simulink library "ammclib_bam_S32K3xx"  (R2016a)
(part 15 of 50)

      |     warning(['Parameter u16NShift_D of ' gcb ' exceeds the fixed-point range.']);
      |   end
      |   u16NShift_Q=ceil(log2(abs(cc1fq)));
      |   tmpsh=ceil(log2(abs(cc2fq)));
      |   if u16NShift_Q<tmpsh
      |     u16NShift_Q=tmpsh;
      |   end
      |   if u16NShift_Q<0
      |     u16NShift_Q=0;
      |   end
      |   if u16NShift_Q>31
      |     u16NShift_Q=31;
      |     warning(['Parameter u16NShift_Q of ' gcb ' exceeds the fixed-point range.']);
      |   end
      |   f32CC1sc_D=round(cc1fd*2^(-u16NShift_D)*2^31);
      |   if f32CC1sc_D>2^31-1
      |     f32CC1sc_D=2^31-1;
      |     warning(['Parameter f32CC1sc_D of ' gcb ' exceeds the fixed-point range.']);
      |   end
      |   if f32CC1sc_D<-2^31
      |     f32CC1sc_D=-2^31;
      |     warning(['Parameter f32CC1sc_D of ' gcb ' exceeds the fixed-point range.']);
      |   end
      |   f32CC2sc_D=round(cc2fd*2^(-u16NShift_D)*2^31);
      |   if f32CC2sc_D>2^31-1
      |     f32CC2sc_D=2^31-1;
      |     warning(['Parameter f32CC2sc_D of ' gcb ' exceeds the fixed-point range.']);
      |   end
      |   if f32CC2sc_D<-2^31
      |     f32CC2sc_D=-2^31;
      |     warning(['Parameter f32CC2sc_D of ' gcb ' exceeds the fixed-point range.']);
      |   end
      |   f32CC1sc_Q=round(cc1fq*2^(-u16NShift_Q)*2^31);
      |   if f32CC1sc_Q>2^31-1
      |     f32CC1sc_Q=2^31-1;
      |     warning(['Parameter f32CC1sc_Q of ' gcb ' exceeds the fixed-point range.']);
      |   end
      |   if f32CC1sc_Q<-2^31
      |     f32CC1sc_Q=-2^31;
      |     warning(['Parameter f32CC1sc_Q of ' gcb ' exceeds the fixed-point range.']);
      |   end
      |   f32CC2sc_Q=round(cc2fq*2^(-u16NShift_Q)*2^31);
      |   if f32CC2sc_Q>2^31-1
      |     f32CC2sc_Q=2^31-1;
      |     warning(['Parameter f32CC2sc_Q of ' gcb ' exceeds the fixed-point range.']);
      |   end
      |   if f32CC2sc_Q<-2^31
      |     f32CC2sc_Q=-2^31;
      |     warning(['Parameter f32CC2sc_Q of ' gcb ' exceeds the fixed-point range.']);
      |   end
      |   if isnan(f32CC1sc_D)
      |     if ~strcmp(f32CC1sc_D_bkup,'0')
      |       set_param(gcb,'f32CC1sc_D','0');
      |     end
      |   else
      |     tmps=num2str(f32CC1sc_D);
      |     if ~strcmp(f32CC1sc_D_bkup,tmps)
      |       set_param(gcb,'f32CC1sc_D',tmps);
      |     end
      |   end
      |   if isnan(f32CC2sc_D)
      |     if ~strcmp(f32CC2sc_D_bkup,'0')
      |       set_param(gcb,'f32CC2sc_D','0');
      |     end
      |   else
      |     tmps=num2str(f32CC2sc_D);
      |     if ~strcmp(f32CC2sc_D_bkup,tmps)
      |       set_param(gcb,'f32CC2sc_D',tmps);
      |     end
      |   end
      |   if isnan(u16NShift_D)
      |     if ~strcmp(u16NShift_D_bkup,'0')
      |       set_param(gcb,'u16NShift_D','0');
      |     end
      |   else
      |     tmps=num2str(u16NShift_D);
      |     if ~strcmp(u16NShift_D_bkup,tmps)
      |       set_param(gcb,'u16NShift_D',tmps);
      |     end
      |   end
      |   if isnan(f32CC1sc_Q)
      |     if ~strcmp(f32CC1sc_Q_bkup,'0')
      |       set_param(gcb,'f32CC1sc_Q','0');
      |     end
      |   else
      |     tmps=num2str(f32CC1sc_Q);
      |     if ~strcmp(f32CC1sc_Q_bkup,tmps)
      |       set_param(gcb,'f32CC1sc_Q',tmps);
      |     end
      |   end
      |   if isnan(f32CC2sc_Q)
      |     if ~strcmp(f32CC2sc_Q_bkup,'0')
      |       set_param(gcb,'f32CC2sc_Q','0');
      |     end
      |   else
      |     tmps=num2str(f32CC2sc_Q);
      |     if ~strcmp(f32CC2sc_Q_bkup,tmps)
      |       set_param(gcb,'f32CC2sc_Q',tmps);
      |     end
      |   end
      |   if isnan(u16NShift_Q)
      |     if ~strcmp(u16NShift_Q_bkup,'0')
      |       set_param(gcb,'u16NShift_Q','0');
      |     end
      |   else
      |     tmps=num2str(u16NShift_Q);
      |     if ~strcmp(u16NShift_Q_bkup,tmps)
      |       set_param(gcb,'u16NShift_Q',tmps);
      |     end
      |   end
      | end
      mask Callback iscale:
      | autoCalcEn=get_param(gcb,'autoCalcEn');
      | if strcmp(autoCalcEn,'on')
      |   SampleTime=Simulink.data.evalinGlobal(bdroot,get_param(gcb,'SampleTime'));
      |   if (SampleTime==-1)
      |     SampleTime=str2double(get_param(gcb,'SampleTime_1'));
      |   end
      |   f32CC1sc_D_bkup=get_param(gcb,'f32CC1sc_D');
      |   f32CC2sc_D_bkup=get_param(gcb,'f32CC2sc_D');
      |   u16NShift_D_bkup=get_param(gcb,'u16NShift_D');
      |   f32CC1sc_Q_bkup=get_param(gcb,'f32CC1sc_Q');
      |   f32CC2sc_Q_bkup=get_param(gcb,'f32CC2sc_Q');
      |   u16NShift_Q_bkup=get_param(gcb,'u16NShift_Q');
      |   intmethod=get_param(gcb,'intmethod');
      |   if0=Simulink.data.evalinGlobal(bdroot,get_param(gcb,'if0'));
      |   iksi=Simulink.data.evalinGlobal(bdroot,get_param(gcb,'iksi'));
      |   Ld=Simulink.data.evalinGlobal(bdroot,get_param(gcb,'Ld'));
      |   Lq=Simulink.data.evalinGlobal(bdroot,get_param(gcb,'Lq'));
      |   Rs=Simulink.data.evalinGlobal(bdroot,get_param(gcb,'Rs'));
      |   uscale=Simulink.data.evalinGlobal(bdroot,get_param(gcb,'uscale'));
      |   iscale=Simulink.data.evalinGlobal(bdroot,get_param(gcb,'iscale'));
      |   if (if0<=0)
      |     warning('Natural frequency f0 must be positive.');
      |   end
      |   if (iksi<=0)
      |     warning('Current loop attenuation must be positive.');
      |   end
      |   if (iksi>1)
      |     warning('Current loop attenuation must not exceed 1.');
      |   end
      |   if (Ld<=0)
      |     warning('Inductance Ld must be positive.');
      |   end
      |   if (Lq<=0)
      |     warning('Inductance Lq must be positive.');
      |   end
      |   if (Rs<0)
      |     warning('Resistance Rs must be non-negative.');
      |   end
      |   if (uscale<=0)
      |     warning('U_max must be positive.');
      |   end
      |   if (iscale<=0)
      |     warning('I_max must be positive.');
      |   end
      |   w0=6.283185307179586*if0;
      |   pgainD=2.0*iksi*w0*Ld-Rs;
      |   igainD=w0*w0*Ld;
      |   pgainQ=2.0*iksi*w0*Lq-Rs;
      |   igainQ=w0*w0*Lq;
      |   if strcmp(intmethod,'Forward Rectangular')
      |     cc1d=pgainD;
      |     cc2d=-pgainD+igainD*SampleTime;
      |     cc1q=pgainQ;
      |     cc2q=-pgainQ+igainQ*SampleTime;
      |   else
      |     if strcmp(intmethod,'Backward Rectangular')
      |       cc1d=pgainD+igainD*SampleTime;
      |       cc2d=-pgainD;
      |       cc1q=pgainQ+igainQ*SampleTime;
      |       cc2q=-pgainQ;
      |     else
      |       cc1d=pgainD+igainD*SampleTime*0.5;
      |       cc2d=-pgainD+igainD*SampleTime*0.5;
      |       cc1q=pgainQ+igainQ*SampleTime*0.5;
      |       cc2q=-pgainQ+igainQ*SampleTime*0.5;
      |     end
      |   end
      |   cc1fd=cc1d*iscale/uscale;
      |   cc2fd=cc2d*iscale/uscale;
      |   cc1fq=cc1q*iscale/uscale;
      |   cc2fq=cc2q*iscale/uscale;
      |   u16NShift_D=ceil(log2(abs(cc1fd)));
      |   tmpsh=ceil(log2(abs(cc2fd)));
      |   if u16NShift_D<tmpsh
      |     u16NShift_D=tmpsh;
      |   end
      |   if u16NShift_D<0
      |     u16NShift_D=0;
      |   end
      |   if u16NShift_D>31
      |     u16NShift_D=31;
      |     warning(['Parameter u16NShift_D of ' gcb ' exceeds the fixed-point range.']);
      |   end
      |   u16NShift_Q=ceil(log2(abs(cc1fq)));
      |   tmpsh=ceil(log2(abs(cc2fq)));
      |   if u16NShift_Q<tmpsh
      |     u16NShift_Q=tmpsh;
      |   end
      |   if u16NShift_Q<0
      |     u16NShift_Q=0;
      |   end
      |   if u16NShift_Q>31
      |     u16NShift_Q=31;
      |     warning(['Parameter u16NShift_Q of ' gcb ' exceeds the fixed-point range.']);
      |   end
      |   f32CC1sc_D=round(cc1fd*2^(-u16NShift_D)*2^31);
      |   if f32CC1sc_D>2^31-1
      |     f32CC1sc_D=2^31-1;
      |     warning(['Parameter f32CC1sc_D of ' gcb ' exceeds the fixed-point range.']);
      |   end
      |   if f32CC1sc_D<-2^31
      |     f32CC1sc_D=-2^31;
      |     warning(['Parameter f32CC1sc_D of ' gcb ' exceeds the fixed-point range.']);
      |   end
      |   f32CC2sc_D=round(cc2fd*2^(-u16NShift_D)*2^31);
      |   if f32CC2sc_D>2^31-1
      |     f32CC2sc_D=2^31-1;
      |     warning(['Parameter f32CC2sc_D of ' gcb ' exceeds the fixed-point range.']);
      |   end
      |   if f32CC2sc_D<-2^31
      |     f32CC2sc_D=-2^31;
      |     warning(['Parameter f32CC2sc_D of ' gcb ' exceeds the fixed-point range.']);
      |   end
      |   f32CC1sc_Q=round(cc1fq*2^(-u16NShift_Q)*2^31);
      |   if f32CC1sc_Q>2^31-1
      |     f32CC1sc_Q=2^31-1;
      |     warning(['Parameter f32CC1sc_Q of ' gcb ' exceeds the fixed-point range.']);
      |   end
      |   if f32CC1sc_Q<-2^31
      |     f32CC1sc_Q=-2^31;
      |     warning(['Parameter f32CC1sc_Q of ' gcb ' exceeds the fixed-point range.']);
      |   end
      |   f32CC2sc_Q=round(cc2fq*2^(-u16NShift_Q)*2^31);
      |   if f32CC2sc_Q>2^31-1
      |     f32CC2sc_Q=2^31-1;
      |     warning(['Parameter f32CC2sc_Q of ' gcb ' exceeds the fixed-point range.']);
      |   end
      |   if f32CC2sc_Q<-2^31
      |     f32CC2sc_Q=-2^31;
      |     warning(['Parameter f32CC2sc_Q of ' gcb ' exceeds the fixed-point range.']);
      |   end
      |   if isnan(f32CC1sc_D)
      |     if ~strcmp(f32CC1sc_D_bkup,'0')
      |       set_param(gcb,'f32CC1sc_D','0');
      |     end
      |   else
      |     tmps=num2str(f32CC1sc_D);
      |     if ~strcmp(f32CC1sc_D_bkup,tmps)
      |       set_param(gcb,'f32CC1sc_D',tmps);
      |     end
      |   end
      |   if isnan(f32CC2sc_D)
      |     if ~strcmp(f32CC2sc_D_bkup,'0')
      |       set_param(gcb,'f32CC2sc_D','0');
      |     end
      |   else
      |     tmps=num2str(f32CC2sc_D);
      |     if ~strcmp(f32CC2sc_D_bkup,tmps)
      |       set_param(gcb,'f32CC2sc_D',tmps);
      |     end
      |   end
      |   if isnan(u16NShift_D)
      |     if ~strcmp(u16NShift_D_bkup,'0')
      |       set_param(gcb,'u16NShift_D','0');
      |     end
      |   else
      |     tmps=num2str(u16NShift_D);
      |     if ~strcmp(u16NShift_D_bkup,tmps)
      |       set_param(gcb,'u16NShift_D',tmps);
      |     end
      |   end
      |   if isnan(f32CC1sc_Q)
      |     if ~strcmp(f32CC1sc_Q_bkup,'0')
      |       set_param(gcb,'f32CC1sc_Q','0');
      |     end
      |   else
      |     tmps=num2str(f32CC1sc_Q);
      |     if ~strcmp(f32CC1sc_Q_bkup,tmps)
      |       set_param(gcb,'f32CC1sc_Q',tmps);
      |     end
      |   end
      |   if isnan(f32CC2sc_Q)
      |     if ~strcmp(f32CC2sc_Q_bkup,'0')
      |       set_param(gcb,'f32CC2sc_Q','0');
      |     end
      |   else
      |     tmps=num2str(f32CC2sc_Q);
      |     if ~strcmp(f32CC2sc_Q_bkup,tmps)
      |       set_param(gcb,'f32CC2sc_Q',tmps);
      |     end
      |   end
      |   if isnan(u16NShift_Q)
      |     if ~strcmp(u16NShift_Q_bkup,'0')
      |       set_param(gcb,'u16NShift_Q','0');
      |     end
      |   else
      |     tmps=num2str(u16NShift_Q);
      |     if ~strcmp(u16NShift_Q_bkup,tmps)
      |       set_param(gcb,'u16NShift_Q',tmps);
      |     end
      |   end
      | end
      mask Callback autoCalcEn:
      | maskStr=get_param(gcb,'showStates');
      | if strcmp(maskStr,'Hide (faster execution)')
      |   p=Simulink.Mask.get(gcb);
      |   autoCalcEn=get_param(gcb,'autoCalcEn');
      |   hintText=p.getDialogControl('timeHint');
      |   if strcmp(autoCalcEn,'on')
      |     param=p.getParameter('iscale');
      |     if strcmp(param.Enabled,'off')
      |       SampleTime=Simulink.data.evalinGlobal(bdroot,get_param(gcb,'SampleTime'));
      |       if SampleTime==-1
      |         SampleTime=str2double(get_param(gcb,'SampleTime_1'));
      |         if isnan(SampleTime)
      |           hintText.Prompt=['Note: Implementation parameters cannot be calculated yet because the block''s inherited sample time is unknown. Simulink will update the sample time when you run the simulation.'];
      |         else
      |           hintText.Prompt=['Caution: Implementation parameters depend on inherited sample time. Make sure that the sample time of the block''s inputs corresponds to the sampling period in the target application.'];
      |         end
      |       else
      |         hintText.Prompt='Caution: Implementation parameters depend on the sample time. Make sure that the simulation time step corresponds to the sampling period in the target application.';
      |       end
      |       p=Simulink.Mask.get(gcb);
      |       param=p.getParameter('intmethod');
      |       param.set('Enabled','on');
      |       param=p.getParameter('if0');
      |       param.set('Enabled','on');
      |       param=p.getParameter('iksi');
      |       param.set('Enabled','on');
      |       param=p.getParameter('Ld');
      |       param.set('Enabled','on');
      |       param=p.getParameter('Lq');
      |       param.set('Enabled','on');
      |       param=p.getParameter('Rs');
      |       param.set('Enabled','on');
      |       param=p.getParameter('uscale');
      |       param.set('Enabled','on');
      |       param=p.getParameter('iscale');
      |       param.set('Enabled','on');
      |     else
      |       SampleTime=Simulink.data.evalinGlobal(bdroot,get_param(gcb,'SampleTime'));
      |       if SampleTime==-1
      |         SampleTime=str2double(get_param(gcb,'SampleTime_1'));
      |       end
      |     end
      |     f32CC1sc_D_bkup=get_param(gcb,'f32CC1sc_D');
      |     f32CC2sc_D_bkup=get_param(gcb,'f32CC2sc_D');
      |     u16NShift_D_bkup=get_param(gcb,'u16NShift_D');
      |     f32CC1sc_Q_bkup=get_param(gcb,'f32CC1sc_Q');
      |     f32CC2sc_Q_bkup=get_param(gcb,'f32CC2sc_Q');
      |     u16NShift_Q_bkup=get_param(gcb,'u16NShift_Q');
      |     intmethod=get_param(gcb,'intmethod');
      |     if0=Simulink.data.evalinGlobal(bdroot,get_param(gcb,'if0'));
      |     iksi=Simulink.data.evalinGlobal(bdroot,get_param(gcb,'iksi'));
      |     Ld=Simulink.data.evalinGlobal(bdroot,get_param(gcb,'Ld'));
      |     Lq=Simulink.data.evalinGlobal(bdroot,get_param(gcb,'Lq'));
      |     Rs=Simulink.data.evalinGlobal(bdroot,get_param(gcb,'Rs'));
      |     uscale=Simulink.data.evalinGlobal(bdroot,get_param(gcb,'uscale'));
      |     iscale=Simulink.data.evalinGlobal(bdroot,get_param(gcb,'iscale'));
      |     if (if0<=0)
      |       warning('Natural frequency f0 must be positive.');
      |     end
      |     if (iksi<=0)
      |       warning('Current loop attenuation must be positive.');
      |     end
      |     if (iksi>1)
      |       warning('Current loop attenuation must not exceed 1.');
      |     end
      |     if (Ld<=0)
      |       warning('Inductance Ld must be positive.');
      |     end
      |     if (Lq<=0)
      |       warning('Inductance Lq must be positive.');
      |     end
      |     if (Rs<0)
      |       warning('Resistance Rs must be non-negative.');
      |     end
      |     if (uscale<=0)
      |       warning('U_max must be positive.');
      |     end
      |     if (iscale<=0)
      |       warning('I_max must be positive.');
      |     end
      |     w0=6.283185307179586*if0;
      |     pgainD=2.0*iksi*w0*Ld-Rs;
      |     igainD=w0*w0*Ld;
      |     pgainQ=2.0*iksi*w0*Lq-Rs;
      |     igainQ=w0*w0*Lq;
      |     if strcmp(intmethod,'Forward Rectangular')
      |       cc1d=pgainD;
      |       cc2d=-pgainD+igainD*SampleTime;
      |       cc1q=pgainQ;
      |       cc2q=-pgainQ+igainQ*SampleTime;
      |     else
      |       if strcmp(intmethod,'Backward Rectangular')
      |         cc1d=pgainD+igainD*SampleTime;
      |         cc2d=-pgainD;
      |         cc1q=pgainQ+igainQ*SampleTime;
      |         cc2q=-pgainQ;
      |       else
      |         cc1d=pgainD+igainD*SampleTime*0.5;
      |         cc2d=-pgainD+igainD*SampleTime*0.5;
      |         cc1q=pgainQ+igainQ*SampleTime*0.5;
      |         cc2q=-pgainQ+igainQ*SampleTime*0.5;
      |       end
      |     end
      |     cc1fd=cc1d*iscale/uscale;
      |     cc2fd=cc2d*iscale/uscale;
      |     cc1fq=cc1q*iscale/uscale;
      |     cc2fq=cc2q*iscale/uscale;
      |     u16NShift_D=ceil(log2(abs(cc1fd)));
      |     tmpsh=ceil(log2(abs(cc2fd)));
      |     if u16NShift_D<tmpsh
      |       u16NShift_D=tmpsh;
      |     end
      |     if u16NShift_D<0
      |       u16NShift_D=0;
      |     end
      |     if u16NShift_D>31
      |       u16NShift_D=31;
      |       warning(['Parameter u16NShift_D of ' gcb ' exceeds the fixed-point range.']);
      |     end
      |     u16NShift_Q=ceil(log2(abs(cc1fq)));
      |     tmpsh=ceil(log2(abs(cc2fq)));
      |     if u16NShift_Q<tmpsh
      |       u16NShift_Q=tmpsh;
      |     end
      |     if u16NShift_Q<0
      |       u16NShift_Q=0;
      |     end
      |     if u16NShift_Q>31
      |       u16NShift_Q=31;
      |       warning(['Parameter u16NShift_Q of ' gcb ' exceeds the fixed-point range.']);
      |     end
      |     f32CC1sc_D=round(cc1fd*2^(-u16NShift_D)*2^31);
      |     if f32CC1sc_D>2^31-1
      |       f32CC1sc_D=2^31-1;
      |       warning(['Parameter f32CC1sc_D of ' gcb ' exceeds the fixed-point range.']);
      |     end
      |     if f32CC1sc_D<-2^31
      |       f32CC1sc_D=-2^31;
      |       warning(['Parameter f32CC1sc_D of ' gcb ' exceeds the fixed-point range.']);
      |     end
      |     f32CC2sc_D=round(cc2fd*2^(-u16NShift_D)*2^31);
      |     if f32CC2sc_D>2^31-1
      |       f32CC2sc_D=2^31-1;
      |       warning(['Parameter f32CC2sc_D of ' gcb ' exceeds the fixed-point range.']);
      |     end
      |     if f32CC2sc_D<-2^31
      |       f32CC2sc_D=-2^31;
      |       warning(['Parameter f32CC2sc_D of ' gcb ' exceeds the fixed-point range.']);
      |     end
      |     f32CC1sc_Q=round(cc1fq*2^(-u16NShift_Q)*2^31);
      |     if f32CC1sc_Q>2^31-1
      |       f32CC1sc_Q=2^31-1;
      |       warning(['Parameter f32CC1sc_Q of ' gcb ' exceeds the fixed-point range.']);
      |     end
      |     if f32CC1sc_Q<-2^31
      |       f32CC1sc_Q=-2^31;
      |       warning(['Parameter f32CC1sc_Q of ' gcb ' exceeds the fixed-point range.']);
      |     end
      |     f32CC2sc_Q=round(cc2fq*2^(-u16NShift_Q)*2^31);
      |     if f32CC2sc_Q>2^31-1
      |       f32CC2sc_Q=2^31-1;
      |       warning(['Parameter f32CC2sc_Q of ' gcb ' exceeds the fixed-point range.']);
      |     end
      |     if f32CC2sc_Q<-2^31
      |       f32CC2sc_Q=-2^31;
      |       warning(['Parameter f32CC2sc_Q of ' gcb ' exceeds the fixed-point range.']);
      |     end
      |     if isnan(f32CC1sc_D)
      |       if ~strcmp(f32CC1sc_D_bkup,'0')
      |         set_param(gcb,'f32CC1sc_D','0');
      |       end
      |     else
      |       tmps=num2str(f32CC1sc_D);
      |       if ~strcmp(f32CC1sc_D_bkup,tmps)
      |         set_param(gcb,'f32CC1sc_D',tmps);
      |       end
      |     end
      |     if isnan(f32CC2sc_D)
      |       if ~strcmp(f32CC2sc_D_bkup,'0')
      |         set_param(gcb,'f32CC2sc_D','0');
      |       end
      |     else
      |       tmps=num2str(f32CC2sc_D);
      |       if ~strcmp(f32CC2sc_D_bkup,tmps)
      |         set_param(gcb,'f32CC2sc_D',tmps);
      |       end
      |     end
      |     if isnan(u16NShift_D)
      |       if ~strcmp(u16NShift_D_bkup,'0')
      |         set_param(gcb,'u16NShift_D','0');
      |       end
      |     else
      |       tmps=num2str(u16NShift_D);
      |       if ~strcmp(u16NShift_D_bkup,tmps)
      |         set_param(gcb,'u16NShift_D',tmps);
      |       end
      |     end
      |     if isnan(f32CC1sc_Q)
      |       if ~strcmp(f32CC1sc_Q_bkup,'0')
      |         set_param(gcb,'f32CC1sc_Q','0');
      |       end
      |     else
      |       tmps=num2str(f32CC1sc_Q);
      |       if ~strcmp(f32CC1sc_Q_bkup,tmps)
      |         set_param(gcb,'f32CC1sc_Q',tmps);
      |       end
      |     end
      |     if isnan(f32CC2sc_Q)
      |       if ~strcmp(f32CC2sc_Q_bkup,'0')
      |         set_param(gcb,'f32CC2sc_Q','0');
      |       end
      |     else
      |       tmps=num2str(f32CC2sc_Q);
      |       if ~strcmp(f32CC2sc_Q_bkup,tmps)
      |         set_param(gcb,'f32CC2sc_Q',tmps);
      |       end
      |     end
      |     if isnan(u16NShift_Q)
      |       if ~strcmp(u16NShift_Q_bkup,'0')
      |         set_param(gcb,'u16NShift_Q','0');
      |       end
      |     else
      |       tmps=num2str(u16NShift_Q);
      |       if ~strcmp(u16NShift_Q_bkup,tmps)
      |         set_param(gcb,'u16NShift_Q',tmps);
      |       end
      |     end
      |   else
      |     param=p.getParameter('iscale');
      |     if strcmp(param.Enabled,'on')
      |       hintText.Prompt='Caution: Implementation parameters are fixed.';
      |       p=Simulink.Mask.get(gcb);
      |       param=p.getParameter('intmethod');
      |       param.set('Enabled','off');
      |       param=p.getParameter('if0');
      |       param.set('Enabled','off');
      |       param=p.getParameter('iksi');
      |       param.set('Enabled','off');
      |       param=p.getParameter('Ld');
      |       param.set('Enabled','off');
      |       param=p.getParameter('Lq');
      |       param.set('Enabled','off');
      |       param=p.getParameter('Rs');
      |       param.set('Enabled','off');
      |       param=p.getParameter('uscale');
      |       param.set('Enabled','off');
      |       param=p.getParameter('iscale');
      |       param.set('Enabled','off');
      |     end
      |   end
      | end
      mask DialogControl CompBut Prompt: Recalculate sample times
      mask DialogControl CompBut Tooltip: Simulink updates the sample times of all blocks when the simulation is run. This button will update the sample times now.
      mask DialogControl CompBut Callback:
      | btn=questdlg('This will apply all changes in all open dialog boxes and update the schematic. Do you want to proceed?','Apply all changes','Continue','Cancel','Continue');
      | if strcmp(btn,'Continue')
      |   dlgs=DAStudio.ToolRoot.getOpenDialogs;
      |   for i=1:length(dlgs)
      |     dlgs(i).apply;
      |   end
      |   try
      |     SampleTime_1=str2double(get_param(gcb,'SampleTime_1'));
      |     ts=Simulink.Block.getSampleTimes(gcb);
      |     ts=ts(1).Value(1);
      |     if (SampleTime_1 ~= ts)
      |       SampleTime_1=ts;
      |       set_param(gcb,'SampleTime_1',num2str(ts));
      |       autoCalcEn=get_param(gcb,'autoCalcEn');
      |       if strcmp(autoCalcEn,'on')
      |         SampleTime=Simulink.data.evalinGlobal(bdroot,get_param(gcb,'SampleTime'));
      |         p=Simulink.Mask.get(gcb);
      |         hintText=p.getDialogControl('timeHint');
      |         if SampleTime==-1
      |           SampleTime=SampleTime_1;
      |           hintText.Prompt='Caution: Implementation parameters depend on inherited sample time. Make sure that the sample time of the block''s inputs corresponds to the sampling period in the target application.';
      |         else
      |           hintText.Prompt='Caution: Implementation parameters depend on the sample time. Make sure that the simulation time step corresponds to the sampling period in the target application.';
      |         end
      |         f32CC1sc_D_bkup=get_param(gcb,'f32CC1sc_D');
      |         f32CC2sc_D_bkup=get_param(gcb,'f32CC2sc_D');
      |         u16NShift_D_bkup=get_param(gcb,'u16NShift_D');
      |         f32CC1sc_Q_bkup=get_param(gcb,'f32CC1sc_Q');
      |         f32CC2sc_Q_bkup=get_param(gcb,'f32CC2sc_Q');
      |         u16NShift_Q_bkup=get_param(gcb,'u16NShift_Q');
      |         intmethod=get_param(gcb,'intmethod');
      |         if0=Simulink.data.evalinGlobal(bdroot,get_param(gcb,'if0'));
      |         iksi=Simulink.data.evalinGlobal(bdroot,get_param(gcb,'iksi'));
      |         Ld=Simulink.data.evalinGlobal(bdroot,get_param(gcb,'Ld'));
      |         Lq=Simulink.data.evalinGlobal(bdroot,get_param(gcb,'Lq'));
      |         Rs=Simulink.data.evalinGlobal(bdroot,get_param(gcb,'Rs'));
      |         uscale=Simulink.data.evalinGlobal(bdroot,get_param(gcb,'uscale'));
      |         iscale=Simulink.data.evalinGlobal(bdroot,get_param(gcb,'iscale'));
      |         if (if0<=0)
      |           warning('Natural frequency f0 must be positive.');
      |         end
      |         if (iksi<=0)
      |           warning('Current loop attenuation must be positive.');
      |         end
      |         if (iksi>1)
      |           warning('Current loop attenuation must not exceed 1.');
      |         end
      |         if (Ld<=0)
      |           warning('Inductance Ld must be positive.');
      |         end
      |         if (Lq<=0)
      |           warning('Inductance Lq must be positive.');
      |         end
      |         if (Rs<0)
      |           warning('Resistance Rs must be non-negative.');
      |         end
      |         if (uscale<=0)
      |           warning('U_max must be positive.');
      |         end
      |         if (iscale<=0)
      |           warning('I_max must be positive.');
      |         end
      |         w0=6.283185307179586*if0;
      |         pgainD=2.0*iksi*w0*Ld-Rs;
      |         igainD=w0*w0*Ld;
      |         pgainQ=2.0*iksi*w0*Lq-Rs;
      |         igainQ=w0*w0*Lq;
      |         if strcmp(intmethod,'Forward Rectangular')
      |           cc1d=pgainD;
      |           cc2d=-pgainD+igainD*SampleTime;
      |           cc1q=pgainQ;
      |           cc2q=-pgainQ+igainQ*SampleTime;
      |         else
      |           if strcmp(intmethod,'Backward Rectangular')
      |             cc1d=pgainD+igainD*SampleTime;
      |             cc2d=-pgainD;
      |             cc1q=pgainQ+igainQ*SampleTime;
      |             cc2q=-pgainQ;
      |           else
      |             cc1d=pgainD+igainD*SampleTime*0.5;
      |             cc2d=-pgainD+igainD*SampleTime*0.5;
      |             cc1q=pgainQ+igainQ*SampleTime*0.5;
      |             cc2q=-pgainQ+igainQ*SampleTime*0.5;
      |           end
      |         end
      |         cc1fd=cc1d*iscale/uscale;
      |         cc2fd=cc2d*iscale/uscale;
      |         cc1fq=cc1q*iscale/uscale;
      |         cc2fq=cc2q*iscale/uscale;
      |         u16NShift_D=ceil(log2(abs(cc1fd)));
      |         tmpsh=ceil(log2(abs(cc2fd)));
      |         if u16NShift_D<tmpsh
      |           u16NShift_D=tmpsh;
      |         end
      |         if u16NShift_D<0
      |           u16NShift_D=0;
      |         end
      |         if u16NShift_D>31
      |           u16NShift_D=31;
      |           warning(['Parameter u16NShift_D of ' gcb ' exceeds the fixed-point range.']);
      |         end
      |         u16NShift_Q=ceil(log2(abs(cc1fq)));
      |         tmpsh=ceil(log2(abs(cc2fq)));
      |         if u16NShift_Q<tmpsh
      |           u16NShift_Q=tmpsh;
      |         end
      |         if u16NShift_Q<0
      |           u16NShift_Q=0;
      |         end
      |         if u16NShift_Q>31
      |           u16NShift_Q=31;
      |           warning(['Parameter u16NShift_Q of ' gcb ' exceeds the fixed-point range.']);
      |         end
      |         f32CC1sc_D=round(cc1fd*2^(-u16NShift_D)*2^31);
      |         if f32CC1sc_D>2^31-1
      |           f32CC1sc_D=2^31-1;
      |           warning(['Parameter f32CC1sc_D of ' gcb ' exceeds the fixed-point range.']);
      |         end
      |         if f32CC1sc_D<-2^31
      |           f32CC1sc_D=-2^31;
      |           warning(['Parameter f32CC1sc_D of ' gcb ' exceeds the fixed-point range.']);
      |         end
      |         f32CC2sc_D=round(cc2fd*2^(-u16NShift_D)*2^31);
      |         if f32CC2sc_D>2^31-1
      |           f32CC2sc_D=2^31-1;
      |           warning(['Parameter f32CC2sc_D of ' gcb ' exceeds the fixed-point range.']);
      |         end
      |         if f32CC2sc_D<-2^31
      |           f32CC2sc_D=-2^31;
      |           warning(['Parameter f32CC2sc_D of ' gcb ' exceeds the fixed-point range.']);
      |         end
      |         f32CC1sc_Q=round(cc1fq*2^(-u16NShift_Q)*2^31);
      |         if f32CC1sc_Q>2^31-1
      |           f32CC1sc_Q=2^31-1;
      |           warning(['Parameter f32CC1sc_Q of ' gcb ' exceeds the fixed-point range.']);
      |         end
      |         if f32CC1sc_Q<-2^31
      |           f32CC1sc_Q=-2^31;
      |           warning(['Parameter f32CC1sc_Q of ' gcb ' exceeds the fixed-point range.']);
      |         end
      |         f32CC2sc_Q=round(cc2fq*2^(-u16NShift_Q)*2^31);
      |         if f32CC2sc_Q>2^31-1
      |           f32CC2sc_Q=2^31-1;
      |           warning(['Parameter f32CC2sc_Q of ' gcb ' exceeds the fixed-point range.']);
      |         end
      |         if f32CC2sc_Q<-2^31
      |           f32CC2sc_Q=-2^31;
      |           warning(['Parameter f32CC2sc_Q of ' gcb ' exceeds the fixed-point range.']);
      |         end
      |         if isnan(f32CC1sc_D)
      |           if ~strcmp(f32CC1sc_D_bkup,'0')
      |             set_param(gcb,'f32CC1sc_D','0');
      |           end
      |         else
      |           tmps=num2str(f32CC1sc_D);
      |           if ~strcmp(f32CC1sc_D_bkup,tmps)
      |             set_param(gcb,'f32CC1sc_D',tmps);
      |           end
      |         end
      |         if isnan(f32CC2sc_D)
      |           if ~strcmp(f32CC2sc_D_bkup,'0')
      |             set_param(gcb,'f32CC2sc_D','0');
      |           end
      |         else
      |           tmps=num2str(f32CC2sc_D);
      |           if ~strcmp(f32CC2sc_D_bkup,tmps)
      |             set_param(gcb,'f32CC2sc_D',tmps);
      |           end
      |         end
      |         if isnan(u16NShift_D)
      |           if ~strcmp(u16NShift_D_bkup,'0')
      |             set_param(gcb,'u16NShift_D','0');
      |           end
      |         else
      |           tmps=num2str(u16NShift_D);
      |           if ~strcmp(u16NShift_D_bkup,tmps)
      |             set_param(gcb,'u16NShift_D',tmps);
      |           end
      |         end
      |         if isnan(f32CC1sc_Q)
      |           if ~strcmp(f32CC1sc_Q_bkup,'0')
      |             set_param(gcb,'f32CC1sc_Q','0');
      |           end
      |         else
      |           tmps=num2str(f32CC1sc_Q);
      |           if ~strcmp(f32CC1sc_Q_bkup,tmps)
      |             set_param(gcb,'f32CC1sc_Q',tmps);
      |           end
      |         end
      |         if isnan(f32CC2sc_Q)
      |           if ~strcmp(f32CC2sc_Q_bkup,'0')
      |             set_param(gcb,'f32CC2sc_Q','0');
      |           end
      |         else
      |           tmps=num2str(f32CC2sc_Q);
      |           if ~strcmp(f32CC2sc_Q_bkup,tmps)
      |             set_param(gcb,'f32CC2sc_Q',tmps);
      |           end
      |         end
      |         if isnan(u16NShift_Q)
      |           if ~strcmp(u16NShift_Q_bkup,'0')
      |             set_param(gcb,'u16NShift_Q','0');
      |           end
      |         else
      |           tmps=num2str(u16NShift_Q);
      |           if ~strcmp(u16NShift_Q_bkup,tmps)
      |             set_param(gcb,'u16NShift_Q',tmps);
      |           end
      |         end
      |       end
      |     end
      |   catch
      |    warning(['Sample time cannot be calculated for the block ' gcb])
      |   end
      | end
      mask DialogControl timeHint Prompt: Note: Implementation parameters cannot be calculated yet because the block's inherited sample time is unknown. Simulink will update the sample time when you run the simulation.
      mask Display:
      | color('black');
      | pos = get_param(gcb, 'Position');
      | width = pos(3) - pos(1);
      | height = pos(4) - pos(2);
      | tX=width/2;
      | tY=height - 25;
      | color('black');
      | text(tX,tY, 'AMCLIB_CurrentLoop_F32', 'horizontalAlignment', 'center');
      | if showStates == 2
      |   color('red');
      |   text(tX,tY - 20, ['debugging mode' char(13) char(10) '(limited performance)'], 'horizontalAlignment', 'center');
      | end
  AMCLIB_FWSpeedLoop_F32 : Subsystem  StartFcn=|  TreatAsAtomicUnit=on  mask(AMCLIB_FWSpeedLoop_F32){showStates=Hide (faster execution), resetStatesEnable=Pre-set according to the first set of inputs after reset, showDebugOutputs=Hide, f32State_Out_showOutput=off, SampleTime=-1, wf0=30, wksi=1, J=1.6e-5, Kt=0.067, lambdaW=0.9, lambdaFW=0.9, Idmax=-5, ramprpm=6, mechspeed=3000, polepairs=1, uscale=15, iscale=10, autoCalcEn=on, u16NSamplesW=0, u16NSamplesFW=0, f32PropGainQ=0, f32IntegGainQ=0, s16PropGainShiftQ=0, s16IntegGainShiftQ=0, f32LowerLimitQ=0, f32UpperLimitQ=0, f32PropGainFW=0, f32IntegGainFW=0, s16PropGainShiftFW=0, s16IntegGainShiftFW=0, f32LowerLimitFW=0, f32UpperLimitFW=0, f32RampUp=0, f32RampDown=0, SampleTime_1=NaN}
      | ts=get_param(gcb,'CompiledSampleTime');
      | if iscell(ts)
      |   ts=ts{1};
      |   if iscell(ts)
      |     ts=ts{1};
      |   end
      | end
      | ts=ts(1);
      | set_param(gcb,'SampleTime_1',num2str(ts));
      | p=Simulink.Mask.get(gcb);
      | hintText=p.getDialogControl('timeHint');
      | SampleTime=Simulink.data.evalinGlobal(bdroot,get_param(gcb,'SampleTime'));
      | p=Simulink.Mask.get(gcb);
      | autoCalcEn=get_param(gcb,'autoCalcEn');
      | if strcmp(autoCalcEn,'on')
      |   if SampleTime==-1
      |     hintText.Prompt='Caution: Implementation parameters depend on inherited sample time. Make sure that the sample time of the block''s inputs corresponds to the sampling period in the target application.';
      |   else
      |     hintText.Prompt='Caution: Implementation parameters depend on the sample time. Make sure that the simulation time step corresponds to the sampling period in the target application.';
      |   end
      |   SampleTime=ts;
      |   u16NSamplesW_bkup=get_param(gcb,'u16NSamplesW');
      |   u16NSamplesFW_bkup=get_param(gcb,'u16NSamplesFW');
      |   f32PropGainQ_bkup=get_param(gcb,'f32PropGainQ');
      |   f32IntegGainQ_bkup=get_param(gcb,'f32IntegGainQ');
      |   s16PropGainShiftQ_bkup=get_param(gcb,'s16PropGainShiftQ');
      |   s16IntegGainShiftQ_bkup=get_param(gcb,'s16IntegGainShiftQ');
      |   f32LowerLimitQ_bkup=get_param(gcb,'f32LowerLimitQ');
      |   f32UpperLimitQ_bkup=get_param(gcb,'f32UpperLimitQ');
      |   f32PropGainFW_bkup=get_param(gcb,'f32PropGainFW');
      |   f32IntegGainFW_bkup=get_param(gcb,'f32IntegGainFW');
      |   s16PropGainShiftFW_bkup=get_param(gcb,'s16PropGainShiftFW');
      |   s16IntegGainShiftFW_bkup=get_param(gcb,'s16IntegGainShiftFW');
      |   f32LowerLimitFW_bkup=get_param(gcb,'f32LowerLimitFW');
      |   f32UpperLimitFW_bkup=get_param(gcb,'f32UpperLimitFW');
      |   f32RampUp_bkup=get_param(gcb,'f32RampUp');
      |   f32RampDown_bkup=get_param(gcb,'f32RampDown');
      |   wf0=Simulink.data.evalinGlobal(bdroot,get_param(gcb,'wf0'));
      |   wksi=Simulink.data.evalinGlobal(bdroot,get_param(gcb,'wksi'));
      |   J=Simulink.data.evalinGlobal(bdroot,get_param(gcb,'J'));
      |   Kt=Simulink.data.evalinGlobal(bdroot,get_param(gcb,'Kt'));
      |   lambdaW=Simulink.data.evalinGlobal(bdroot,get_param(gcb,'lambdaW'));
      |   lambdaFW=Simulink.data.evalinGlobal(bdroot,get_param(gcb,'lambdaFW'));
      |   Idmax=Simulink.data.evalinGlobal(bdroot,get_param(gcb,'Idmax'));
      |   ramprpm=Simulink.data.evalinGlobal(bdroot,get_param(gcb,'ramprpm'));
      |   mechspeed=Simulink.data.evalinGlobal(bdroot,get_param(gcb,'mechspeed'));
      |   polepairs=Simulink.data.evalinGlobal(bdroot,get_param(gcb,'polepairs'));
      |   uscale=Simulink.data.evalinGlobal(bdroot,get_param(gcb,'uscale'));
      |   iscale=Simulink.data.evalinGlobal(bdroot,get_param(gcb,'iscale'));
      |   if (wf0<=0)
      |     warning('Natural frequency f0 must be positive.');
      |   end
      |   if (wksi<=0)
      |     warning('Current loop attenuation must be positive.');
      |   end
      |   if (wksi>1)
      |     warning('Current loop attenuation must not exceed 1.');
      |   end
      |   if (J<=0)
      |     warning('Moment of inertia J must be positive.');
      |   end
      |   if (Kt<=0)
      |     warning('Torque constant Kt must be positive.');
      |   end
      |   if (lambdaW<0)
      |     warning('MA filter smoothing factor must be in the range 0..1.');
      |   end
      |   if (lambdaW>1)
      |     warning('MA filter smoothing factor must be in the range 0..1.');
      |   end
      |   if (lambdaFW<0)
      |     warning('MA filter smoothing factor must be in the range 0..1.');
      |   end
      |   if (lambdaFW>1)
      |     warning('MA filter smoothing factor must be in the range 0..1.');
      |   end
      |   if (mechspeed<=0)
      |     warning('Max. speed must be positive.');
      |   end
      |   if (polepairs<1)
      |     warning('Number of pole pairs must be a natural number (1, 2, 3, ...).');
      |   end
      |   if (round(polepairs)~=polepairs)
      |     warning('Number of pole pairs must be a natural number (1, 2, 3, ...).');
      |   end
      |   if (uscale<=0)
      |     warning('U_max must be positive.');
      |   end
      |   if (iscale<=0)
      |     warning('I_max must be positive.');
      |   end
      |   w0=6.283185307179586*wf0;
      |   pgain=2.0*wksi*w0*J/Kt;
      |   igain=w0*w0*J/Kt;
      |   wmax=polepairs*mechspeed*0.1047197551196598;
      |   kpf=pgain*wmax/iscale;
      |   s16PropGainShiftQ=ceil(log2(abs(kpf)));
      |   if s16PropGainShiftQ<-31
      |     s16PropGainShiftQ=-31;
      |   end
      |   if s16PropGainShiftQ>31
      |     s16PropGainShiftQ=31;
      |     warning(['Parameter s16PropGainShiftQ of ' gcb ' exceeds the fixed-point range.']);
      |   end
      |   f32PropGainQ=round(kpf*2^(-s16PropGainShiftQ)*2^31);
      |   if f32PropGainQ>2^31-1
      |     f32PropGainQ=2^31-1;
      |     warning(['Parameter f32PropGainQ of ' gcb ' exceeds the fixed-point range.']);
      |   end
      |   if f32PropGainQ<-2^31
      |     f32PropGainQ=-2^31;
      |     warning(['Parameter f32PropGainQ of ' gcb ' exceeds the fixed-point range.']);
      |   end
      |   kif=igain*SampleTime*0.5*wmax/iscale;
      |   s16IntegGainShiftQ=ceil(log2(abs(kif)));
      |   if s16IntegGainShiftQ<-31
      |     s16IntegGainShiftQ=-31;
      |   end
      |   if s16IntegGainShiftQ>31
      |     s16IntegGainShiftQ=31;
      |     warning(['Parameter s16IntegGainShiftQ of ' gcb ' exceeds the fixed-point range.']);
      |   end
      |   f32IntegGainQ=round(kif*2^(-s16IntegGainShiftQ)*2^31);
      |   if f32IntegGainQ>2^31-1
      |     f32IntegGainQ=2^31-1;
      |     warning(['Parameter f32IntegGainQ of ' gcb ' exceeds the fixed-point range.']);
      |   end
      |   if f32IntegGainQ<-2^31
      |     f32IntegGainQ=-2^31;
      |     warning(['Parameter f32IntegGainQ of ' gcb ' exceeds the fixed-point range.']);
      |   end
      |   f32LowerLimitQ=-2147483648;
      |   f32UpperLimitQ=2147483647;
      |   fwkpf=0.9*pgain*wmax/iscale;
      |   s16PropGainShiftFW=ceil(log2(abs(fwkpf)));
      |   if s16PropGainShiftFW<-31
      |     s16PropGainShiftFW=-31;
      |   end
      |   if s16PropGainShiftFW>31
      |     s16PropGainShiftFW=31;
      |     warning(['Parameter s16PropGainShiftFW of ' gcb ' exceeds the fixed-point range.']);
      |   end
      |   f32PropGainFW=round(fwkpf*2^(-s16PropGainShiftFW)*2^31);
      |   if f32PropGainFW>2^31-1
      |     f32PropGainFW=2^31-1;
      |     warning(['Parameter f32PropGainFW of ' gcb ' exceeds the fixed-point range.']);
      |   end
      |   if f32PropGainFW<-2^31
      |     f32PropGainFW=-2^31;
      |     warning(['Parameter f32PropGainFW of ' gcb ' exceeds the fixed-point range.']);
      |   end
      |   s16IntegGainShiftFW=s16IntegGainShiftQ;
      |   f32IntegGainFW=f32IntegGainQ;
      |   if (Idmax<0)
      |     iratio=abs(Idmax)/iscale;
      |     if (abs(iratio) > 1)
      |       iratio = 0;
      |     end
      |     lowlim=0.3183098861837907*acos(iratio)-0.5;
      |   else
      |     lowlim=0.0;
      |   end
      |   f32LowerLimitFW=round(lowlim*2^31);
      |   if f32LowerLimitFW>2^31-1
      |     f32LowerLimitFW=2^31-1;
      |     warning(['Parameter f32LowerLimitFW of ' gcb ' exceeds the fixed-point range.']);
      |   end
      |   if f32LowerLimitFW<-2^31
      |     f32LowerLimitFW=-2^31;
      |     warning(['Parameter f32LowerLimitFW of ' gcb ' exceeds the fixed-point range.']);
      |   end
      |   f32UpperLimitFW=0;
      |   u16NSamplesW=round(log2(1.0/abs(lambdaW)));
      |   if u16NSamplesW>31
      |     u16NSamplesW=31;
      |   end
      |   if u16NSamplesW<0
      |     u16NSamplesW=0;
      |   end
      |   u16NSamplesFW=round(log2(1.0/abs(lambdaFW)));
      |   if u16NSamplesFW>31
      |     u16NSamplesFW=31;
      |   end
      |   if u16NSamplesFW<0
      |     u16NSamplesFW=0;
      |   end
      |   rampsc=polepairs*abs(ramprpm)*0.1047197551196598/wmax;
      |   f32RampUp=round(rampsc*2^31);
      |   if f32RampUp>2^31-1
      |     f32RampUp=2^31-1;
      |     warning(['Parameter f32RampUp of ' gcb ' exceeds the fixed-point range.']);
      |   end
      |   if f32RampUp<-2^31
      |     f32RampUp=-2^31;
      |     warning(['Parameter f32RampUp of ' gcb ' exceeds the fixed-point range.']);
      |   end
      |   f32RampDown=round(rampsc*2^31);
      |   if f32RampDown>2^31-1
      |     f32RampDown=2^31-1;
      |     warning(['Parameter f32RampDown of ' gcb ' exceeds the fixed-point range.']);
      |   end
      |   if f32RampDown<-2^31
      |     f32RampDown=-2^31;
      |     warning(['Parameter f32RampDown of ' gcb ' exceeds the fixed-point range.']);
      |   end
      |   if isnan(u16NSamplesW)
      |     if ~strcmp(u16NSamplesW_bkup,'0')
      |       set_param(gcb,'u16NSamplesW','0');
      |     end
      |   else
      |     tmps=num2str(u16NSamplesW);
      |     if ~strcmp(u16NSamplesW_bkup,tmps)
      |       set_param(gcb,'u16NSamplesW',tmps);
      |     end
      |   end
      |   if isnan(u16NSamplesFW)
      |     if ~strcmp(u16NSamplesFW_bkup,'0')
      |       set_param(gcb,'u16NSamplesFW','0');
      |     end
      |   else
      |     tmps=num2str(u16NSamplesFW);
      |     if ~strcmp(u16NSamplesFW_bkup,tmps)
      |       set_param(gcb,'u16NSamplesFW',tmps);
      |     end
      |   end
      |   if isnan(f32PropGainQ)
      |     if ~strcmp(f32PropGainQ_bkup,'0')
      |       set_param(gcb,'f32PropGainQ','0');
      |     end
      |   else
      |     tmps=num2str(f32PropGainQ);
      |     if ~strcmp(f32PropGainQ_bkup,tmps)
      |       set_param(gcb,'f32PropGainQ',tmps);
      |     end
      |   end
      |   if isnan(f32IntegGainQ)
      |     if ~strcmp(f32IntegGainQ_bkup,'0')
      |       set_param(gcb,'f32IntegGainQ','0');
      |     end
      |   else
      |     tmps=num2str(f32IntegGainQ);
      |     if ~strcmp(f32IntegGainQ_bkup,tmps)
      |       set_param(gcb,'f32IntegGainQ',tmps);
      |     end
      |   end
      |   if isnan(s16PropGainShiftQ)
      |     if ~strcmp(s16PropGainShiftQ_bkup,'0')
      |       set_param(gcb,'s16PropGainShiftQ','0');
      |     end
      |   else
      |     tmps=num2str(s16PropGainShiftQ);
      |     if ~strcmp(s16PropGainShiftQ_bkup,tmps)
      |       set_param(gcb,'s16PropGainShiftQ',tmps);
      |     end
      |   end
      |   if isnan(s16IntegGainShiftQ)
      |     if ~strcmp(s16IntegGainShiftQ_bkup,'0')
      |       set_param(gcb,'s16IntegGainShiftQ','0');
      |     end
      |   else
      |     tmps=num2str(s16IntegGainShiftQ);
      |     if ~strcmp(s16IntegGainShiftQ_bkup,tmps)
      |       set_param(gcb,'s16IntegGainShiftQ',tmps);
      |     end
      |   end
      |   if isnan(f32LowerLimitQ)
      |     if ~strcmp(f32LowerLimitQ_bkup,'0')
      |       set_param(gcb,'f32LowerLimitQ','0');
      |     end
      |   else
      |     tmps=num2str(f32LowerLimitQ);
      |     if ~strcmp(f32LowerLimitQ_bkup,tmps)
      |       set_param(gcb,'f32LowerLimitQ',tmps);
      |     end
      |   end
      |   if isnan(f32UpperLimitQ)
      |     if ~strcmp(f32UpperLimitQ_bkup,'0')
      |       set_param(gcb,'f32UpperLimitQ','0');
      |     end
      |   else
      |     tmps=num2str(f32UpperLimitQ);
      |     if ~strcmp(f32UpperLimitQ_bkup,tmps)
      |       set_param(gcb,'f32UpperLimitQ',tmps);
      |     end
      |   end
      |   if isnan(f32PropGainFW)
      |     if ~strcmp(f32PropGainFW_bkup,'0')
      |       set_param(gcb,'f32PropGainFW','0');
      |     end
      |   else
      |     tmps=num2str(f32PropGainFW);
      |     if ~strcmp(f32PropGainFW_bkup,tmps)
      |       set_param(gcb,'f32PropGainFW',tmps);
      |     end
      |   end
      |   if isnan(f32IntegGainFW)
      |     if ~strcmp(f32IntegGainFW_bkup,'0')
      |       set_param(gcb,'f32IntegGainFW','0');
      |     end
      |   else
      |     tmps=num2str(f32IntegGainFW);
      |     if ~strcmp(f32IntegGainFW_bkup,tmps)
      |       set_param(gcb,'f32IntegGainFW',tmps);
      |     end
      |   end
      |   if isnan(s16PropGainShiftFW)
      |     if ~strcmp(s16PropGainShiftFW_bkup,'0')
      |       set_param(gcb,'s16PropGainShiftFW','0');
      |     end
      |   else
      |     tmps=num2str(s16PropGainShiftFW);
      |     if ~strcmp(s16PropGainShiftFW_bkup,tmps)
      |       set_param(gcb,'s16PropGainShiftFW',tmps);
      |     end
      |   end
      |   if isnan(s16IntegGainShiftFW)
      |     if ~strcmp(s16IntegGainShiftFW_bkup,'0')
      |       set_param(gcb,'s16IntegGainShiftFW','0');
      |     end
      |   else
      |     tmps=num2str(s16IntegGainShiftFW);
      |     if ~strcmp(s16IntegGainShiftFW_bkup,tmps)
      |       set_param(gcb,'s16IntegGainShiftFW',tmps);
      |     end
      |   end
      |   if isnan(f32LowerLimitFW)
      |     if ~strcmp(f32LowerLimitFW_bkup,'0')
      |       set_param(gcb,'f32LowerLimitFW','0');
      |     end
      |   else
      |     tmps=num2str(f32LowerLimitFW);
      |     if ~strcmp(f32LowerLimitFW_bkup,tmps)
      |       set_param(gcb,'f32LowerLimitFW',tmps);
      |     end
      |   end
      |   if isnan(f32UpperLimitFW)
      |     if ~strcmp(f32UpperLimitFW_bkup,'0')
      |       set_param(gcb,'f32UpperLimitFW','0');
      |     end
      |   else
      |     tmps=num2str(f32UpperLimitFW);
      |     if ~strcmp(f32UpperLimitFW_bkup,tmps)
      |       set_param(gcb,'f32UpperLimitFW',tmps);
      |     end
      |   end
      |   if isnan(f32RampUp)
      |     if ~strcmp(f32RampUp_bkup,'0')
      |       set_param(gcb,'f32RampUp','0');
      |     end
      |   else
      |     tmps=num2str(f32RampUp);
      |     if ~strcmp(f32RampUp_bkup,tmps)
      |       set_param(gcb,'f32RampUp',tmps);
      |     end
      |   end
      |   if isnan(f32RampDown)
      |     if ~strcmp(f32RampDown_bkup,'0')
      |       set_param(gcb,'f32RampDown','0');
      |     end
      |   else
      |     tmps=num2str(f32RampDown);
      |     if ~strcmp(f32RampDown_bkup,tmps)
      |       set_param(gcb,'f32RampDown',tmps);
      |     end
      |   end
      | end
      mask prompts: showStates "Show internal states:"; resetStatesEnable "Internal state after reset:"; showDebugOutputs "Show debugging outputs:"; f32State_Out_showOutput "Output speed ramp state (f32State_Out)"; SampleTime "Sample time (-1 for inherited):"; wf0 "Speed loop natural frequency f0 [Hz]:"; wksi "Speed loop attenuation ξ:"; J "Moment of inertia J [kg*m^2]:"; Kt "Motor torque constant Kt [N*m/A]:"; lambdaW "Speed MA filter smoothing factor λ (0..1):"; lambdaFW "Field weakening MA filter smoothing factor λ (0..1):"; Idmax "Maximum negative d-axis current (demagnetization current - CAUTION!) [A]:"; ramprpm "Speed ramp slope [ΔRPM per speed loop iteration]:"; mechspeed "Maximum mechanical speed of the motor [RPM]:"; polepairs "Number of pole pairs of the motor:"; uscale "U_max (maximum DC bus voltage) [V]:"; iscale "I_max (maximum phase current) [A]:"; autoCalcEn "Calculate implementation parameters from physical parameters"; u16NSamplesW "u16NSamplesW (velocity GDFLIB_FilterMA - recalculated smoothing factor):"; u16NSamplesFW "u16NSamplesFW (FW GDFLIB_FilterMA - recalculated smoothing factor):"; f32PropGainQ "f32PropGainQ (q-axis GFLIB_ControllerPIpAW - proportional gain):"; f32IntegGainQ "f32IntegGainQ (q-axis GFLIB_ControllerPIpAW - integral gain):"; s16PropGainShiftQ "s16PropGainShiftQ (q-axis GFLIB_ControllerPIpAW - scaling bitwise shift applied to the proportional gain):"; s16IntegGainShiftQ "s16IntegGainShiftQ (q-axis GFLIB_ControllerPIpAW - scaling bitwise shift applied to the integral gain):"; f32LowerLimitQ "f32LowerLimitQ (q-axis GFLIB_ControllerPIpAW - lower limit):"; f32UpperLimitQ "f32UpperLimitQ (q-axis GFLIB_ControllerPIpAW - upper limit):"; f32PropGainFW "f32PropGainFW (FW GFLIB_ControllerPIpAW - proportional gain):"; f32IntegGainFW "f32IntegGainFW (FW GFLIB_ControllerPIpAW - integral gain):"; s16PropGainShiftFW "s16PropGainShiftFW (FW GFLIB_ControllerPIpAW - scaling bitwise shift applied to the proportional gain):"; s16IntegGainShiftFW "s16IntegGainShiftFW (FW GFLIB_ControllerPIpAW - scaling bitwise shift applied to the integral gain):"; f32LowerLimitFW "f32LowerLimitFW (FW GFLIB_ControllerPIpAW - lower limit):"; f32UpperLimitFW "f32UpperLimitFW (FW GFLIB_ControllerPIpAW - upper limit):"; f32RampUp "f32RampUp (Ramp up increment coefficient):"; f32RampDown "f32RampDown (Ramp decrement coefficient):"; SampleTime_1 "Discrete sample time:"
      mask help: Speed loop controller with Field Weakening capability for the PMSM field-oriented control algorithm in 32-bit fixed-point fractional implementation. This block supports re-initialization of the internal state during simulation. If the block is reset, the outputs of the MA filters, PI controllers, and the ramp will be aligned with the inputs f32FilterMAWOut_preset, f32FilterMAFWOut_preset, f32ControllerPIpAWQOut_preset, f32ControllerPIpAWFWOut_preset, and f32RampOut_preset. Refer to the AMMCLIB User's Guide for further details.
      mask init:
      | ddName = get_param(bdroot,'DataDictionary');
      | if length(ddName)==0
      |   set_param(bdroot,'DataDictionary','ammclib_types.sldd');
      | else
      |   dd = Simulink.data.dictionary.open(ddName);
      |   data = getSection(dd,'Design Data');
      |   if ~exist(data,'SWLIBS_2Syst_F16')
      |     addDataSource(dd,'ammclib_types.sldd');
      |     saveChanges(dd);
      |   end
      | end
      | outputsChanged = 0;
      | 
      | if showStates == 1
      |   % hidden state variables
      |   if strcmp(get_param([gcb '/u16NSamplesW'], 'BlockType'), 'Inport')
      |     posblk = get_param(gcb, 'Position');
      | 
      |     pos = get_param([gcb, '/u16NSamplesW'], 'Position');
      |     orient = get_param([gcb, '/u16NSamplesW'], 'Orientation');
      |     delete_block([gcb, '/u16NSamplesW']);
      |     add_block('built-in/Ground', [gcb, '/u16NSamplesW'], 'Position', pos, 'Orientation', orient);
      | 
      |     pos = get_param([gcb, '/u16NSamplesFW'], 'Position');
      |     orient = get_param([gcb, '/u16NSamplesFW'], 'Orientation');
      |     delete_block([gcb, '/u16NSamplesFW']);
      |     add_block('built-in/Ground', [gcb, '/u16NSamplesFW'], 'Position', pos, 'Orientation', orient);
      | 
      |     pos = get_param([gcb, '/f32PropGainQ'], 'Position');
      |     orient = get_param([gcb, '/f32PropGainQ'], 'Orientation');
      |     delete_block([gcb, '/f32PropGainQ']);
      |     add_block('built-in/Ground', [gcb, '/f32PropGainQ'], 'Position', pos, 'Orientation', orient);
      | 
      |     pos = get_param([gcb, '/f32IntegGainQ'], 'Position');
      |     orient = get_param([gcb, '/f32IntegGainQ'], 'Orientation');
      |     delete_block([gcb, '/f32IntegGainQ']);
      |     add_block('built-in/Ground', [gcb, '/f32IntegGainQ'], 'Position', pos, 'Orientation', orient);
      | 
      |     pos = get_param([gcb, '/s16PropGainShiftQ'], 'Position');
      |     orient = get_param([gcb, '/s16PropGainShiftQ'], 'Orientation');
      |     delete_block([gcb, '/s16PropGainShiftQ']);
      |     add_block('built-in/Ground', [gcb, '/s16PropGainShiftQ'], 'Position', pos, 'Orientation', orient);
      | 
      |     pos = get_param([gcb, '/s16IntegGainShiftQ'], 'Position');
      |     orient = get_param([gcb, '/s16IntegGainShiftQ'], 'Orientation');
      |     delete_block([gcb, '/s16IntegGainShiftQ']);
      |     add_block('built-in/Ground', [gcb, '/s16IntegGainShiftQ'], 'Position', pos, 'Orientation', orient);
      | 
      |     pos = get_param([gcb, '/f32LowerLimitQ'], 'Position');
      |     orient = get_param([gcb, '/f32LowerLimitQ'], 'Orientation');
      |     delete_block([gcb, '/f32LowerLimitQ']);
      |     add_block('built-in/Ground', [gcb, '/f32LowerLimitQ'], 'Position', pos, 'Orientation', orient);
      | 
      |     pos = get_param([gcb, '/f32UpperLimitQ'], 'Position');
      |     orient = get_param([gcb, '/f32UpperLimitQ'], 'Orientation');
      |     delete_block([gcb, '/f32UpperLimitQ']);
      |     add_block('built-in/Ground', [gcb, '/f32UpperLimitQ'], 'Position', pos, 'Orientation', orient);
      | 
      |     pos = get_param([gcb, '/f32PropGainFW'], 'Position');
      |     orient = get_param([gcb, '/f32PropGainFW'], 'Orientation');
      |     delete_block([gcb, '/f32PropGainFW']);
      |     add_block('built-in/Ground', [gcb, '/f32PropGainFW'], 'Position', pos, 'Orientation', orient);
      | 
      |     pos = get_param([gcb, '/f32IntegGainFW'], 'Position');
      |     orient = get_param([gcb, '/f32IntegGainFW'], 'Orientation');
      |     delete_block([gcb, '/f32IntegGainFW']);
      |     add_block('built-in/Ground', [gcb, '/f32IntegGainFW'], 'Position', pos, 'Orientation', orient);
      | 
      |     pos = get_param([gcb, '/s16PropGainShiftFW'], 'Position');
      |     orient = get_param([gcb, '/s16PropGainShiftFW'], 'Orientation');
      |     delete_block([gcb, '/s16PropGainShiftFW']);
      |     add_block('built-in/Ground', [gcb, '/s16PropGainShiftFW'], 'Position', pos, 'Orientation', orient);
      | 
      |     pos = get_param([gcb, '/s16IntegGainShiftFW'], 'Position');
      |     orient = get_param([gcb, '/s16IntegGainShiftFW'], 'Orientation');
      |     delete_block([gcb, '/s16IntegGainShiftFW']);
      |     add_block('built-in/Ground', [gcb, '/s16IntegGainShiftFW'], 'Position', pos, 'Orientation', orient);
      | 
      |     pos = get_param([gcb, '/f32LowerLimitFW'], 'Position');
      |     orient = get_param([gcb, '/f32LowerLimitFW'], 'Orientation');
      |     delete_block([gcb, '/f32LowerLimitFW']);
      |     add_block('built-in/Ground', [gcb, '/f32LowerLimitFW'], 'Position', pos, 'Orientation', orient);
      | 
      |     pos = get_param([gcb, '/f32UpperLimitFW'], 'Position');
      |     orient = get_param([gcb, '/f32UpperLimitFW'], 'Orientation');
      |     delete_block([gcb, '/f32UpperLimitFW']);
      |     add_block('built-in/Ground', [gcb, '/f32UpperLimitFW'], 'Position', pos, 'Orientation', orient);
      | 
      |     pos = get_param([gcb, '/f32RampUp'], 'Position');
      |     orient = get_param([gcb, '/f32RampUp'], 'Orientation');
      |     delete_block([gcb, '/f32RampUp']);
      |     add_block('built-in/Ground', [gcb, '/f32RampUp'], 'Position', pos, 'Orientation', orient);
      | 
      |     pos = get_param([gcb, '/f32RampDown'], 'Position');
      |     orient = get_param([gcb, '/f32RampDown'], 'Orientation');
      |     delete_block([gcb, '/f32RampDown']);
      |     add_block('built-in/Ground', [gcb, '/f32RampDown'], 'Position', pos, 'Orientation', orient);
      | 
      |     pos = get_param([gcb, '/f32IQReqK_1'], 'Position');
      |     orient = get_param([gcb, '/f32IQReqK_1'], 'Orientation');
      |     delete_block([gcb, '/f32IQReqK_1']);
      |     add_block('built-in/Ground', [gcb, '/f32IQReqK_1'], 'Position', pos, 'Orientation', orient);
      | 
      |     pos = get_param([gcb, '/f32AccW'], 'Position');
      |     orient = get_param([gcb, '/f32AccW'], 'Orientation');
      |     delete_block([gcb, '/f32AccW']);
      |     add_block('built-in/Ground', [gcb, '/f32AccW'], 'Position', pos, 'Orientation', orient);
      | 
      |     pos = get_param([gcb, '/f32AccFW'], 'Position');
      |     orient = get_param([gcb, '/f32AccFW'], 'Orientation');
      |     delete_block([gcb, '/f32AccFW']);
      |     add_block('built-in/Ground', [gcb, '/f32AccFW'], 'Position', pos, 'Orientation', orient);
      | 
      |     pos = get_param([gcb, '/f32IntegPartK_1Q'], 'Position');
      |     orient = get_param([gcb, '/f32IntegPartK_1Q'], 'Orientation');
      |     delete_block([gcb, '/f32IntegPartK_1Q']);
      |     add_block('built-in/Ground', [gcb, '/f32IntegPartK_1Q'], 'Position', pos, 'Orientation', orient);
      | 
      |     pos = get_param([gcb, '/f32InK_1Q'], 'Position');
      |     orient = get_param([gcb, '/f32InK_1Q'], 'Orientation');
      |     delete_block([gcb, '/f32InK_1Q']);
      |     add_block('built-in/Ground', [gcb, '/f32InK_1Q'], 'Position', pos, 'Orientation', orient);
      | 
      |     pos = get_param([gcb, '/f32IntegPartK_1FW'], 'Position');
      |     orient = get_param([gcb, '/f32IntegPartK_1FW'], 'Orientation');
      |     delete_block([gcb, '/f32IntegPartK_1FW']);
      |     add_block('built-in/Ground', [gcb, '/f32IntegPartK_1FW'], 'Position', pos, 'Orientation', orient);
      | 
      |     pos = get_param([gcb, '/f32InK_1FW'], 'Position');
      |     orient = get_param([gcb, '/f32InK_1FW'], 'Orientation');
      |     delete_block([gcb, '/f32InK_1FW']);
      |     add_block('built-in/Ground', [gcb, '/f32InK_1FW'], 'Position', pos, 'Orientation', orient);
      | 
      |     pos = get_param([gcb, '/f32State'], 'Position');
      |     orient = get_param([gcb, '/f32State'], 'Orientation');
      |     delete_block([gcb, '/f32State']);
      |     add_block('built-in/Ground', [gcb, '/f32State'], 'Position', pos, 'Orientation', orient);
      | 
      | 
      |     pmask=Simulink.Mask.get(gcb);
      |     pctrl=pmask.getParameter('SampleTime');
      |     pctrl.set('TypeOptions',{'f32VelocityReq/SampleTime','f32VelocityFbck/SampleTime','f32IQFbck/SampleTime','f32UQReq/SampleTime','f32UQLim/SampleTime','f32FilterMAWOut_preset/SampleTime','f32FilterMAFWOut_preset/SampleTime','f32ControllerPIpAWQOut_preset/SampleTime','f32ControllerPIpAWFWOut_preset/SampleTime','f32RampOut_preset/SampleTime'});
      | 
      |     pos = get_param([gcb '/f32AccW_Out'], 'Position');
      |     orient = get_param([gcb '/f32AccW_Out'], 'Orientation');
      |     delete_block([gcb '/f32AccW_Out']);
      |     add_block('built-in/Terminator', [gcb '/f32AccW_Out'], 'Position', pos, 'Orientation', orient);
      | 
      |     pos = get_param([gcb '/f32AccFW_Out'], 'Position');
      |     orient = get_param([gcb '/f32AccFW_Out'], 'Orientation');
      |     delete_block([gcb '/f32AccFW_Out']);
      |     add_block('built-in/Terminator', [gcb '/f32AccFW_Out'], 'Position', pos, 'Orientation', orient);
      | 
      |     pos = get_param([gcb '/f32IntegPartK_1Q_Out'], 'Position');
      |     orient = get_param([gcb '/f32IntegPartK_1Q_Out'], 'Orientation');
      |     delete_block([gcb '/f32IntegPartK_1Q_Out']);
      |     add_block('built-in/Terminator', [gcb '/f32IntegPartK_1Q_Out'], 'Position', pos, 'Orientation', orient);
      | 
      |     pos = get_param([gcb '/f32InK_1Q_Out'], 'Position');
      |     orient = get_param([gcb '/f32InK_1Q_Out'], 'Orientation');
      |     delete_block([gcb '/f32InK_1Q_Out']);
      |     add_block('built-in/Terminator', [gcb '/f32InK_1Q_Out'], 'Position', pos, 'Orientation', orient);
      | 
      |     pos = get_param([gcb '/f32IntegPartK_1FW_Out'], 'Position');
      |     orient = get_param([gcb '/f32IntegPartK_1FW_Out'], 'Orientation');
      |     delete_block([gcb '/f32IntegPartK_1FW_Out']);
      |     add_block('built-in/Terminator', [gcb '/f32IntegPartK_1FW_Out'], 'Position', pos, 'Orientation', orient);
      | 
      |     pos = get_param([gcb '/f32InK_1FW_Out'], 'Position');
      |     orient = get_param([gcb '/f32InK_1FW_Out'], 'Orientation');
      |     delete_block([gcb '/f32InK_1FW_Out']);
      |     add_block('built-in/Terminator', [gcb '/f32InK_1FW_Out'], 'Position', pos, 'Orientation', orient);
      | 
      |     if strcmp(get_param([gcb '/f32WReqFilt'], 'BlockType'), 'Outport')
      |       pos = get_param([gcb '/f32WReqFilt'], 'Position');
      |       orient = get_param([gcb '/f32WReqFilt'], 'Orientation');
      |       delete_block([gcb '/f32WReqFilt']);
      |       add_block('built-in/Terminator', [gcb '/f32WReqFilt'], 'Position', pos, 'Orientation', orient);
      | 
      |       pos = get_param([gcb '/f32WErr'], 'Position');
      |       orient = get_param([gcb '/f32WErr'], 'Orientation');
      |       delete_block([gcb '/f32WErr']);
      |       add_block('built-in/Terminator', [gcb '/f32WErr'], 'Position', pos, 'Orientation', orient);
      | 
      |       pos = get_param([gcb '/f32WFbckFilt'], 'Position');
      |       orient = get_param([gcb '/f32WFbckFilt'], 'Orientation');
      |       delete_block([gcb '/f32WFbckFilt']);
      |       add_block('built-in/Terminator', [gcb '/f32WFbckFilt'], 'Position', pos, 'Orientation', orient);
      | 
      |       pos = get_param([gcb '/f32IDQReqAmp'], 'Position');
      |       orient = get_param([gcb '/f32IDQReqAmp'], 'Orientation');
      |       delete_block([gcb '/f32IDQReqAmp']);
      |       add_block('built-in/Terminator', [gcb '/f32IDQReqAmp'], 'Position', pos, 'Orientation', orient);
      | 
      |       pos = get_param([gcb '/f32IQErrSign'], 'Position');
      |       orient = get_param([gcb '/f32IQErrSign'], 'Orientation');
      |       delete_block([gcb '/f32IQErrSign']);
      |       add_block('built-in/Terminator', [gcb '/f32IQErrSign'], 'Position', pos, 'Orientation', orient);
      | 
      |       pos = get_param([gcb '/f32IQErr'], 'Position');
      |       orient = get_param([gcb '/f32IQErr'], 'Orientation');
      |       delete_block([gcb '/f32IQErr']);
      |       add_block('built-in/Terminator', [gcb '/f32IQErr'], 'Position', pos, 'Orientation', orient);
      | 
      |       pos = get_param([gcb '/f32FWErr'], 'Position');
      |       orient = get_param([gcb '/f32FWErr'], 'Orientation');
      |       delete_block([gcb '/f32FWErr']);
      |       add_block('built-in/Terminator', [gcb '/f32FWErr'], 'Position', pos, 'Orientation', orient);
      | 
      |       pos = get_param([gcb '/f32UQErr'], 'Position');
      |       orient = get_param([gcb '/f32UQErr'], 'Orientation');
      |       delete_block([gcb '/f32UQErr']);
      |       add_block('built-in/Terminator', [gcb '/f32UQErr'], 'Position', pos, 'Orientation', orient);
      | 
      |       pos = get_param([gcb '/f32FWErrFilt'], 'Position');
      |       orient = get_param([gcb '/f32FWErrFilt'], 'Orientation');
      |       delete_block([gcb '/f32FWErrFilt']);
      |       add_block('built-in/Terminator', [gcb '/f32FWErrFilt'], 'Position', pos, 'Orientation', orient);
      | 
      |       pos = get_param([gcb '/f32FWAngle'], 'Position');
      |       orient = get_param([gcb '/f32FWAngle'], 'Orientation');
      |       delete_block([gcb '/f32FWAngle']);
      |       add_block('built-in/Terminator', [gcb '/f32FWAngle'], 'Position', pos, 'Orientation', orient);
      | 
      |       pos = get_param([gcb '/f32FWSin'], 'Position');
      |       orient = get_param([gcb '/f32FWSin'], 'Orientation');
      |       delete_block([gcb '/f32FWSin']);
      |       add_block('built-in/Terminator', [gcb '/f32FWSin'], 'Position', pos, 'Orientation', orient);
      | 
      |       pos = get_param([gcb '/f32FWCos'], 'Position');
      |       orient = get_param([gcb '/f32FWCos'], 'Orientation');
      |       delete_block([gcb '/f32FWCos']);
      |       add_block('built-in/Terminator', [gcb '/f32FWCos'], 'Position', pos, 'Orientation', orient);
      | 
      |     end
      | 
      |     set_param([gcb '/f32VelocityReq'], 'Port', '1');
      |     set_param([gcb '/f32VelocityFbck'], 'Port', '2');
      |     set_param([gcb '/f32IQFbck'], 'Port', '3');
      |     set_param([gcb '/f32UQReq'], 'Port', '4');
      |     set_param([gcb '/f32UQLim'], 'Port', '5');
      |     set_param([gcb '/f32FilterMAWOut_preset'], 'Port', '6');
      |     set_param([gcb '/f32FilterMAFWOut_preset'], 'Port', '7');
      |     set_param([gcb '/f32ControllerPIpAWQOut_preset'], 'Port', '8');
      |     set_param([gcb '/f32ControllerPIpAWFWOut_preset'], 'Port', '9');
      |     set_param([gcb '/f32RampOut_preset'], 'Port', '10');
      | 
      |     tmpOutCnt=0;
      |     tmpOutCnt=tmpOutCnt+1;
      |     set_param([gcb '/pIDQReq'], 'Port', num2str(tmpOutCnt));
      |     tmpOutCnt=tmpOutCnt+1;
      |     set_param([gcb '/u16LimitFlagQ'], 'Port', num2str(tmpOutCnt));
      |     tmpOutCnt=tmpOutCnt+1;
      |     set_param([gcb '/u16LimitFlagFW'], 'Port', num2str(tmpOutCnt));
      |     if strcmp(get_param([gcb '/f32State_Out'], 'BlockType'), 'Outport')
      |       tmpOutCnt=tmpOutCnt+1;
      |       set_param([gcb '/f32State_Out'], 'Port', num2str(tmpOutCnt));
      |     end
      | 
      |   autoCalcEn=get_param(gcb,'autoCalcEn');
      |   if strcmp(autoCalcEn,'on')
      |     set_param(gcb,'MaskEnables',{'on','on','off','on','on','on','on','on','on','on','on','on','on','on','on','on','on','on','on','on','on','on','on','on','on','on','on','on','on','on','on','on','on','on','off'});
      |   else
      |     set_param(gcb,'MaskEnables',{'on','on','off','on','on','off','off','off','off','off','off','off','off','off','off','off','off','on','on','on','on','on','on','on','on','on','on','on','on','on','on','on','on','on','off'});
      |   end
      | 
      |     if (posblk(4) - posblk(2)) > 275
      |       height = 275;
      |       set_param(gcb,'Position',[posblk(1), posblk(2), posblk(3), posblk(2)+height])
      |     end
      |   end
      | else
      |   % shown state variables
      |   if strcmp(get_param([gcb '/u16NSamplesW'], 'BlockType'), 'Ground')
      |     posblk = get_param(gcb, 'Position');
      | 
      |     pos = get_param([gcb, '/u16NSamplesW'], 'Position');
      |     orient = get_param([gcb, '/u16NSamplesW'], 'Orientation');
      |     delete_block([gcb, '/u16NSamplesW']);
      |     add_block('built-in/Inport', [gcb, '/u16NSamplesW'], 'Position', pos, 'Orientation', orient, 'OutDataTypeStr', 'uint16');
      | 
      |     pos = get_param([gcb, '/u16NSamplesFW'], 'Position');
      |     orient = get_param([gcb, '/u16NSamplesFW'], 'Orientation');
      |     delete_block([gcb, '/u16NSamplesFW']);
      |     add_block('built-in/Inport', [gcb, '/u16NSamplesFW'], 'Position', pos, 'Orientation', orient, 'OutDataTypeStr', 'uint16');
      | 
      |     pos = get_param([gcb, '/f32PropGainQ'], 'Position');
      |     orient = get_param([gcb, '/f32PropGainQ'], 'Orientation');
      |     delete_block([gcb, '/f32PropGainQ']);
      |     add_block('built-in/Inport', [gcb, '/f32PropGainQ'], 'Position', pos, 'Orientation', orient, 'OutDataTypeStr', 'int32');
      | 
      |     pos = get_param([gcb, '/f32IntegGainQ'], 'Position');
      |     orient = get_param([gcb, '/f32IntegGainQ'], 'Orientation');
      |     delete_block([gcb, '/f32IntegGainQ']);
      |     add_block('built-in/Inport', [gcb, '/f32IntegGainQ'], 'Position', pos, 'Orientation', orient, 'OutDataTypeStr', 'int32');
      | 
      |     pos = get_param([gcb, '/s16PropGainShiftQ'], 'Position');
      |     orient = get_param([gcb, '/s16PropGainShiftQ'], 'Orientation');
      |     delete_block([gcb, '/s16PropGainShiftQ']);
      |     add_block('built-in/Inport', [gcb, '/s16PropGainShiftQ'], 'Position', pos, 'Orientation', orient, 'OutDataTypeStr', 'int16');
      | 
      |     pos = get_param([gcb, '/s16IntegGainShiftQ'], 'Position');
      |     orient = get_param([gcb, '/s16IntegGainShiftQ'], 'Orientation');
      |     delete_block([gcb, '/s16IntegGainShiftQ']);
      |     add_block('built-in/Inport', [gcb, '/s16IntegGainShiftQ'], 'Position', pos, 'Orientation', orient, 'OutDataTypeStr', 'int16');
      | 
      |     pos = get_param([gcb, '/f32LowerLimitQ'], 'Position');
      |     orient = get_param([gcb, '/f32LowerLimitQ'], 'Orientation');
      |     delete_block([gcb, '/f32LowerLimitQ']);
      |     add_block('built-in/Inport', [gcb, '/f32LowerLimitQ'], 'Position', pos, 'Orientation', orient, 'OutDataTypeStr', 'int32');
      | 
      |     pos = get_param([gcb, '/f32UpperLimitQ'], 'Position');
      |     orient = get_param([gcb, '/f32UpperLimitQ'], 'Orientation');
      |     delete_block([gcb, '/f32UpperLimitQ']);
      |     add_block('built-in/Inport', [gcb, '/f32UpperLimitQ'], 'Position', pos, 'Orientation', orient, 'OutDataTypeStr', 'int32');
      | 
      |     pos = get_param([gcb, '/f32PropGainFW'], 'Position');
      |     orient = get_param([gcb, '/f32PropGainFW'], 'Orientation');
      |     delete_block([gcb, '/f32PropGainFW']);
      |     add_block('built-in/Inport', [gcb, '/f32PropGainFW'], 'Position', pos, 'Orientation', orient, 'OutDataTypeStr', 'int32');
      | 
      |     pos = get_param([gcb, '/f32IntegGainFW'], 'Position');
      |     orient = get_param([gcb, '/f32IntegGainFW'], 'Orientation');
      |     delete_block([gcb, '/f32IntegGainFW']);
      |     add_block('built-in/Inport', [gcb, '/f32IntegGainFW'], 'Position', pos, 'Orientation', orient, 'OutDataTypeStr', 'int32');
      | 
      |     pos = get_param([gcb, '/s16PropGainShiftFW'], 'Position');
      |     orient = get_param([gcb, '/s16PropGainShiftFW'], 'Orientation');
      |     delete_block([gcb, '/s16PropGainShiftFW']);
      |     add_block('built-in/Inport', [gcb, '/s16PropGainShiftFW'], 'Position', pos, 'Orientation', orient, 'OutDataTypeStr', 'int16');
      | 
      |     pos = get_param([gcb, '/s16IntegGainShiftFW'], 'Position');
      |     orient = get_param([gcb, '/s16IntegGainShiftFW'], 'Orientation');
      |     delete_block([gcb, '/s16IntegGainShiftFW']);
      |     add_block('built-in/Inport', [gcb, '/s16IntegGainShiftFW'], 'Position', pos, 'Orientation', orient, 'OutDataTypeStr', 'int16');
      | 
      |     pos = get_param([gcb, '/f32LowerLimitFW'], 'Position');
      |     orient = get_param([gcb, '/f32LowerLimitFW'], 'Orientation');
      |     delete_block([gcb, '/f32LowerLimitFW']);
      |     add_block('built-in/Inport', [gcb, '/f32LowerLimitFW'], 'Position', pos, 'Orientation', orient, 'OutDataTypeStr', 'int32');
      | 
      |     pos = get_param([gcb, '/f32UpperLimitFW'], 'Position');
      |     orient = get_param([gcb, '/f32UpperLimitFW'], 'Orientation');
      |     delete_block([gcb, '/f32UpperLimitFW']);
      |     add_block('built-in/Inport', [gcb, '/f32UpperLimitFW'], 'Position', pos, 'Orientation', orient, 'OutDataTypeStr', 'int32');
      | 
      |     pos = get_param([gcb, '/f32RampUp'], 'Position');
      |     orient = get_param([gcb, '/f32RampUp'], 'Orientation');
      |     delete_block([gcb, '/f32RampUp']);
      |     add_block('built-in/Inport', [gcb, '/f32RampUp'], 'Position', pos, 'Orientation', orient, 'OutDataTypeStr', 'int32');
      | 
      |     pos = get_param([gcb, '/f32RampDown'], 'Position');
      |     orient = get_param([gcb, '/f32RampDown'], 'Orientation');
      |     delete_block([gcb, '/f32RampDown']);
      |     add_block('built-in/Inport', [gcb, '/f32RampDown'], 'Position', pos, 'Orientation', orient, 'OutDataTypeStr', 'int32');
      | 
      |     pos = get_param([gcb, '/f32IQReqK_1'], 'Position');
      |     orient = get_param([gcb, '/f32IQReqK_1'], 'Orientation');
      |     delete_block([gcb, '/f32IQReqK_1']);
      |     add_block('built-in/Inport', [gcb, '/f32IQReqK_1'], 'Position', pos, 'Orientation', orient, 'OutDataTypeStr', 'int32');
      | 
      |     pos = get_param([gcb, '/f32AccW'], 'Position');
      |     orient = get_param([gcb, '/f32AccW'], 'Orientation');
      |     delete_block([gcb, '/f32AccW']);
      |     add_block('built-in/Inport', [gcb, '/f32AccW'], 'Position', pos, 'Orientation', orient, 'OutDataTypeStr', 'int32');
      | 
      |     pos = get_param([gcb, '/f32AccFW'], 'Position');
      |     orient = get_param([gcb, '/f32AccFW'], 'Orientation');
      |     delete_block([gcb, '/f32AccFW']);
      |     add_block('built-in/Inport', [gcb, '/f32AccFW'], 'Position', pos, 'Orientation', orient, 'OutDataTypeStr', 'int32');
      | 
      |     pos = get_param([gcb, '/f32IntegPartK_1Q'], 'Position');
      |     orient = get_param([gcb, '/f32IntegPartK_1Q'], 'Orientation');
      |     delete_block([gcb, '/f32IntegPartK_1Q']);
      |     add_block('built-in/Inport', [gcb, '/f32IntegPartK_1Q'], 'Position', pos, 'Orientation', orient, 'OutDataTypeStr', 'int32');
      | 
      |     pos = get_param([gcb, '/f32InK_1Q'], 'Position');
      |     orient = get_param([gcb, '/f32InK_1Q'], 'Orientation');
      |     delete_block([gcb, '/f32InK_1Q']);
      |     add_block('built-in/Inport', [gcb, '/f32InK_1Q'], 'Position', pos, 'Orientation', orient, 'OutDataTypeStr', 'int32');
      | 
      |     pos = get_param([gcb, '/f32IntegPartK_1FW'], 'Position');
      |     orient = get_param([gcb, '/f32IntegPartK_1FW'], 'Orientation');
      |     delete_block([gcb, '/f32IntegPartK_1FW']);
      |     add_block('built-in/Inport', [gcb, '/f32IntegPartK_1FW'], 'Position', pos, 'Orientation', orient, 'OutDataTypeStr', 'int32');
      | 
      |     pos = get_param([gcb, '/f32InK_1FW'], 'Position');
      |     orient = get_param([gcb, '/f32InK_1FW'], 'Orientation');
      |     delete_block([gcb, '/f32InK_1FW']);
      |     add_block('built-in/Inport', [gcb, '/f32InK_1FW'], 'Position', pos, 'Orientation', orient, 'OutDataTypeStr', 'int32');
      | 
      |     pos = get_param([gcb, '/f32State'], 'Position');
      |     orient = get_param([gcb, '/f32State'], 'Orientation');
      |     delete_block([gcb, '/f32State']);
      |     add_block('built-in/Inport', [gcb, '/f32State'], 'Position', pos, 'Orientation', orient, 'OutDataTypeStr', 'int32');
      | 
      | 
      | 
      |     pos = get_param([gcb '/f32AccW_Out'], 'Position');
      |     orient = get_param([gcb '/f32AccW_Out'], 'Orientation');
      |     delete_block([gcb '/f32AccW_Out']);
      |     add_block('built-in/Outport', [gcb '/f32AccW_Out'], 'Position', pos, 'Orientation', orient);
      | 
      |     pos = get_param([gcb '/f32AccFW_Out'], 'Position');
      |     orient = get_param([gcb '/f32AccFW_Out'], 'Orientation');
      |     delete_block([gcb '/f32AccFW_Out']);
      |     add_block('built-in/Outport', [gcb '/f32AccFW_Out'], 'Position', pos, 'Orientation', orient);
      | 
      |     pos = get_param([gcb '/f32IntegPartK_1Q_Out'], 'Position');
      |     orient = get_param([gcb '/f32IntegPartK_1Q_Out'], 'Orientation');
      |     delete_block([gcb '/f32IntegPartK_1Q_Out']);
      |     add_block('built-in/Outport', [gcb '/f32IntegPartK_1Q_Out'], 'Position', pos, 'Orientation', orient);
      | 
      |     pos = get_param([gcb '/f32InK_1Q_Out'], 'Position');
      |     orient = get_param([gcb '/f32InK_1Q_Out'], 'Orientation');
      |     delete_block([gcb '/f32InK_1Q_Out']);
      |     add_block('built-in/Outport', [gcb '/f32InK_1Q_Out'], 'Position', pos, 'Orientation', orient);
      | 
      |     pos = get_param([gcb '/f32IntegPartK_1FW_Out'], 'Position');
      |     orient = get_param([gcb '/f32IntegPartK_1FW_Out'], 'Orientation');
      |     delete_block([gcb '/f32IntegPartK_1FW_Out']);
      |     add_block('built-in/Outport', [gcb '/f32IntegPartK_1FW_Out'], 'Position', pos, 'Orientation', orient);
      | 
      |     pos = get_param([gcb '/f32InK_1FW_Out'], 'Position');
      |     orient = get_param([gcb '/f32InK_1FW_Out'], 'Orientation');
      |     delete_block([gcb '/f32InK_1FW_Out']);
      |     add_block('built-in/Outport', [gcb '/f32InK_1FW_Out'], 'Position', pos, 'Orientation', orient);
      | 
      | 
      |     pmask=Simulink.Mask.get(gcb);
      |     pctrl=pmask.getParameter('SampleTime');
      |     pctrl.set('TypeOptions',{'f32VelocityReq/SampleTime','f32VelocityFbck/SampleTime','f32IQFbck/SampleTime','f32UQReq/SampleTime','f32UQLim/SampleTime','f32FilterMAWOut_preset/SampleTime','f32FilterMAFWOut_preset/SampleTime','f32ControllerPIpAWQOut_preset/SampleTime','f32ControllerPIpAWFWOut_preset/SampleTime','f32RampOut_preset/SampleTime','u16NSamplesW/SampleTime','u16NSamplesFW/SampleTime','f32PropGainQ/SampleTime','f32IntegGainQ/SampleTime','s16PropGainShiftQ/SampleTime','s16IntegGainShiftQ/SampleTime','f32LowerLimitQ/SampleTime','f32UpperLimitQ/SampleTime','f32PropGainFW/SampleTime','f32IntegGainFW/SampleTime','s16PropGainShiftFW/SampleTime','s16IntegGainShiftFW/SampleTime','f32LowerLimitFW/SampleTime','f32UpperLimitFW/SampleTime','f32RampUp/SampleTime','f32RampDown/SampleTime','f32IQReqK_1/SampleTime','f32AccW/SampleTime','f32AccFW/SampleTime','f32IntegPartK_1Q/SampleTime','f32InK_1Q/SampleTime','f32IntegPartK_1FW/SampleTime','f32InK_1FW/SampleTime','f32State/SampleTime'});
      | 
      |     if (showDebugOutputs == 2) && (strcmp(get_param([gcb '/f32WReqFilt'], 'BlockType'), 'Terminator'))
      |       pos = get_param([gcb '/f32WReqFilt'], 'Position');
      |       orient = get_param([gcb '/f32WReqFilt'], 'Orientation');
      |       delete_block([gcb '/f32WReqFilt']);
      |       add_block('built-in/Outport', [gcb '/f32WReqFilt'], 'Position', pos, 'Orientation', orient);
      | 
      |       pos = get_param([gcb '/f32WErr'], 'Position');
      |       orient = get_param([gcb '/f32WErr'], 'Orientation');
      |       delete_block([gcb '/f32WErr']);
      |       add_block('built-in/Outport', [gcb '/f32WErr'], 'Position', pos, 'Orientation', orient);
      | 
      |       pos = get_param([gcb '/f32WFbckFilt'], 'Position');
      |       orient = get_param([gcb '/f32WFbckFilt'], 'Orientation');
      |       delete_block([gcb '/f32WFbckFilt']);
      |       add_block('built-in/Outport', [gcb '/f32WFbckFilt'], 'Position', pos, 'Orientation', orient);
      | 
      |       pos = get_param([gcb '/f32IDQReqAmp'], 'Position');
      |       orient = get_param([gcb '/f32IDQReqAmp'], 'Orientation');
      |       delete_block([gcb '/f32IDQReqAmp']);
      |       add_block('built-in/Outport', [gcb '/f32IDQReqAmp'], 'Position', pos, 'Orientation', orient);
      | 
      |       pos = get_param([gcb '/f32IQErrSign'], 'Position');
      |       orient = get_param([gcb '/f32IQErrSign'], 'Orientation');
      |       delete_block([gcb '/f32IQErrSign']);
      |       add_block('built-in/Outport', [gcb '/f32IQErrSign'], 'Position', pos, 'Orientation', orient);
      | 
      |       pos = get_param([gcb '/f32IQErr'], 'Position');
      |       orient = get_param([gcb '/f32IQErr'], 'Orientation');
      |       delete_block([gcb '/f32IQErr']);
      |       add_block('built-in/Outport', [gcb '/f32IQErr'], 'Position', pos, 'Orientation', orient);
      | 
      |       pos = get_param([gcb '/f32FWErr'], 'Position');
      |       orient = get_param([gcb '/f32FWErr'], 'Orientation');
      |       delete_block([gcb '/f32FWErr']);
      |       add_block('built-in/Outport', [gcb '/f32FWErr'], 'Position', pos, 'Orientation', orient);
      | 
      |       pos = get_param([gcb '/f32UQErr'], 'Position');
      |       orient = get_param([gcb '/f32UQErr'], 'Orientation');
      |       delete_block([gcb '/f32UQErr']);
      |       add_block('built-in/Outport', [gcb '/f32UQErr'], 'Position', pos, 'Orientation', orient);
      | 
      |       pos = get_param([gcb '/f32FWErrFilt'], 'Position');
      |       orient = get_param([gcb '/f32FWErrFilt'], 'Orientation');
      |       delete_block([gcb '/f32FWErrFilt']);
      |       add_block('built-in/Outport', [gcb '/f32FWErrFilt'], 'Position', pos, 'Orientation', orient);
      | 
      |       pos = get_param([gcb '/f32FWAngle'], 'Position');
      |       orient = get_param([gcb '/f32FWAngle'], 'Orientation');
      |       delete_block([gcb '/f32FWAngle']);
      |       add_block('built-in/Outport', [gcb '/f32FWAngle'], 'Position', pos, 'Orientation', orient);
      | 
      |       pos = get_param([gcb '/f32FWSin'], 'Position');
      |       orient = get_param([gcb '/f32FWSin'], 'Orientation');
      |       delete_block([gcb '/f32FWSin']);
      |       add_block('built-in/Outport', [gcb '/f32FWSin'], 'Position', pos, 'Orientation', orient);
      | 
      |       pos = get_param([gcb '/f32FWCos'], 'Position');
      |       orient = get_param([gcb '/f32FWCos'], 'Orientation');
      |       delete_block([gcb '/f32FWCos']);
      |       add_block('built-in/Outport', [gcb '/f32FWCos'], 'Position', pos, 'Orientation', orient);
      | 
      |     end
      | 
      |     set_param([gcb '/f32VelocityReq'], 'Port', '1');
      |     set_param([gcb '/f32VelocityFbck'], 'Port', '2');
      |     set_param([gcb '/f32IQFbck'], 'Port', '3');
      |     set_param([gcb '/f32UQReq'], 'Port', '4');
      |     set_param([gcb '/f32UQLim'], 'Port', '5');
      |     set_param([gcb '/f32FilterMAWOut_preset'], 'Port', '6');
      |     set_param([gcb '/f32FilterMAFWOut_preset'], 'Port', '7');
      |     set_param([gcb '/f32ControllerPIpAWQOut_preset'], 'Port', '8');
      |     set_param([gcb '/f32ControllerPIpAWFWOut_preset'], 'Port', '9');
      |     set_param([gcb '/f32RampOut_preset'], 'Port', '10');
      |     set_param([gcb '/u16NSamplesW'], 'Port', '11');
      |     set_param([gcb '/u16NSamplesFW'], 'Port', '12');
      |     set_param([gcb '/f32PropGainQ'], 'Port', '13');
      |     set_param([gcb '/f32IntegGainQ'], 'Port', '14');
      |     set_param([gcb '/s16PropGainShiftQ'], 'Port', '15');
      |     set_param([gcb '/s16IntegGainShiftQ'], 'Port', '16');
      |     set_param([gcb '/f32LowerLimitQ'], 'Port', '17');
      |     set_param([gcb '/f32UpperLimitQ'], 'Port', '18');
      |     set_param([gcb '/f32PropGainFW'], 'Port', '19');
      |     set_param([gcb '/f32IntegGainFW'], 'Port', '20');
      |     set_param([gcb '/s16PropGainShiftFW'], 'Port', '21');
      |     set_param([gcb '/s16IntegGainShiftFW'], 'Port', '22');
      |     set_param([gcb '/f32LowerLimitFW'], 'Port', '23');
      |     set_param([gcb '/f32UpperLimitFW'], 'Port', '24');
      |     set_param([gcb '/f32RampUp'], 'Port', '25');
      |     set_param([gcb '/f32RampDown'], 'Port', '26');
      |     set_param([gcb '/f32IQReqK_1'], 'Port', '27');
      |     set_param([gcb '/f32AccW'], 'Port', '28');
      |     set_param([gcb '/f32AccFW'], 'Port', '29');
      |     set_param([gcb '/f32IntegPartK_1Q'], 'Port', '30');
      |     set_param([gcb '/f32InK_1Q'], 'Port', '31');
      |     set_param([gcb '/f32IntegPartK_1FW'], 'Port', '32');
      |     set_param([gcb '/f32InK_1FW'], 'Port', '33');
      |     set_param([gcb '/f32State'], 'Port', '34');
      | 
      |     if (showDebugOutputs == 2)
      |       tmpOutCnt=0;
      |       tmpOutCnt=tmpOutCnt+1;
      |       set_param([gcb '/pIDQReq'], 'Port', num2str(tmpOutCnt));
      |       tmpOutCnt=tmpOutCnt+1;
      |       set_param([gcb '/u16LimitFlagQ'], 'Port', num2str(tmpOutCnt));
      |       tmpOutCnt=tmpOutCnt+1;
      |       set_param([gcb '/u16LimitFlagFW'], 'Port', num2str(tmpOutCnt));
      |       tmpOutCnt=tmpOutCnt+1;
      |       set_param([gcb '/f32WReqFilt'], 'Port', num2str(tmpOutCnt));
      |       tmpOutCnt=tmpOutCnt+1;
      |       set_param([gcb '/f32WErr'], 'Port', num2str(tmpOutCnt));
      |       tmpOutCnt=tmpOutCnt+1;
      |       set_param([gcb '/f32WFbckFilt'], 'Port', num2str(tmpOutCnt));
      |       tmpOutCnt=tmpOutCnt+1;
      |       set_param([gcb '/f32IDQReqAmp'], 'Port', num2str(tmpOutCnt));
      |       tmpOutCnt=tmpOutCnt+1;
      |       set_param([gcb '/f32IQErrSign'], 'Port', num2str(tmpOutCnt));
      |       tmpOutCnt=tmpOutCnt+1;
      |       set_param([gcb '/f32IQErr'], 'Port', num2str(tmpOutCnt));
      |       tmpOutCnt=tmpOutCnt+1;
      |       set_param([gcb '/f32FWErr'], 'Port', num2str(tmpOutCnt));
      |       tmpOutCnt=tmpOutCnt+1;
      |       set_param([gcb '/f32UQErr'], 'Port', num2str(tmpOutCnt));
      |       tmpOutCnt=tmpOutCnt+1;
      |       set_param([gcb '/f32FWErrFilt'], 'Port', num2str(tmpOutCnt));
      |       tmpOutCnt=tmpOutCnt+1;
      |       set_param([gcb '/f32FWAngle'], 'Port', num2str(tmpOutCnt));
      |       tmpOutCnt=tmpOutCnt+1;
      |       set_param([gcb '/f32FWSin'], 'Port', num2str(tmpOutCnt));
      |       tmpOutCnt=tmpOutCnt+1;
      |       set_param([gcb '/f32FWCos'], 'Port', num2str(tmpOutCnt));
      |       tmpOutCnt=tmpOutCnt+1;
      |       set_param([gcb '/f32AccW_Out'], 'Port', num2str(tmpOutCnt));
      |       tmpOutCnt=tmpOutCnt+1;
      |       set_param([gcb '/f32AccFW_Out'], 'Port', num2str(tmpOutCnt));
      |       tmpOutCnt=tmpOutCnt+1;
      |       set_param([gcb '/f32IntegPartK_1Q_Out'], 'Port', num2str(tmpOutCnt));
      |       tmpOutCnt=tmpOutCnt+1;
      |       set_param([gcb '/f32InK_1Q_Out'], 'Port', num2str(tmpOutCnt));
      |       tmpOutCnt=tmpOutCnt+1;
      |       set_param([gcb '/f32IntegPartK_1FW_Out'], 'Port', num2str(tmpOutCnt));
      |       tmpOutCnt=tmpOutCnt+1;
      |       set_param([gcb '/f32InK_1FW_Out'], 'Port', num2str(tmpOutCnt));
      |       if strcmp(get_param([gcb '/f32State_Out'], 'BlockType'), 'Outport')
      |         tmpOutCnt=tmpOutCnt+1;
      |         set_param([gcb '/f32State_Out'], 'Port', num2str(tmpOutCnt));
      |       end
      |     else
      |       tmpOutCnt=0;
      |       tmpOutCnt=tmpOutCnt+1;
      |       set_param([gcb '/pIDQReq'], 'Port', num2str(tmpOutCnt));
      |       tmpOutCnt=tmpOutCnt+1;
      |       set_param([gcb '/u16LimitFlagQ'], 'Port', num2str(tmpOutCnt));
      |       tmpOutCnt=tmpOutCnt+1;
      |       set_param([gcb '/u16LimitFlagFW'], 'Port', num2str(tmpOutCnt));
      |       tmpOutCnt=tmpOutCnt+1;
      |       set_param([gcb '/f32AccW_Out'], 'Port', num2str(tmpOutCnt));
      |       tmpOutCnt=tmpOutCnt+1;
      |       set_param([gcb '/f32AccFW_Out'], 'Port', num2str(tmpOutCnt));
      |       tmpOutCnt=tmpOutCnt+1;
      |       set_param([gcb '/f32IntegPartK_1Q_Out'], 'Port', num2str(tmpOutCnt));
      |       tmpOutCnt=tmpOutCnt+1;
      |       set_param([gcb '/f32InK_1Q_Out'], 'Port', num2str(tmpOutCnt));
      |       tmpOutCnt=tmpOutCnt+1;
      |       set_param([gcb '/f32IntegPartK_1FW_Out'], 'Port', num2str(tmpOutCnt));
      |       tmpOutCnt=tmpOutCnt+1;
      |       set_param([gcb '/f32InK_1FW_Out'], 'Port', num2str(tmpOutCnt));
      |       if strcmp(get_param([gcb '/f32State_Out'], 'BlockType'), 'Outport')
      |         tmpOutCnt=tmpOutCnt+1;
      |         set_param([gcb '/f32State_Out'], 'Port', num2str(tmpOutCnt));
      |       end
      |     end
      | 
      |     set_param(gcb,'MaskEnables',{'on','on','on','on','on','off','off','off','off','off','off','off','off','off','off','off','off','off','off','off','off','off','off','off','off','off','off','off','off','off','off','off','off','off','off'});
      | 
      |     if (posblk(4) - posblk(2)) < 875
      |       height = 875;
      |       set_param(gcb,'Position',[posblk(1), posblk(2), posblk(3), posblk(2)+height])
      |     end
      |   else
      |     if (showDebugOutputs == 2) && (strcmp(get_param([gcb '/f32WReqFilt'], 'BlockType'), 'Terminator'))
      |       % shown debugging outputs
      |       pos = get_param([gcb '/f32WReqFilt'], 'Position');
      |       orient = get_param([gcb '/f32WReqFilt'], 'Orientation');
      |       delete_block([gcb '/f32WReqFilt']);
      |       add_block('built-in/Outport', [gcb '/f32WReqFilt'], 'Position', pos, 'Orientation', orient);
      | 
      |       pos = get_param([gcb '/f32WErr'], 'Position');
      |       orient = get_param([gcb '/f32WErr'], 'Orientation');
      |       delete_block([gcb '/f32WErr']);
      |       add_block('built-in/Outport', [gcb '/f32WErr'], 'Position', pos, 'Orientation', orient);
      | 
      |       pos = get_param([gcb '/f32WFbckFilt'], 'Position');
      |       orient = get_param([gcb '/f32WFbckFilt'], 'Orientation');
      |       delete_block([gcb '/f32WFbckFilt']);
      |       add_block('built-in/Outport', [gcb '/f32WFbckFilt'], 'Position', pos, 'Orientation', orient);
      | 
      |       pos = get_param([gcb '/f32IDQReqAmp'], 'Position');
      |       orient = get_param([gcb '/f32IDQReqAmp'], 'Orientation');
      |       delete_block([gcb '/f32IDQReqAmp']);
      |       add_block('built-in/Outport', [gcb '/f32IDQReqAmp'], 'Position', pos, 'Orientation', orient);
      | 
      |       pos = get_param([gcb '/f32IQErrSign'], 'Position');
      |       orient = get_param([gcb '/f32IQErrSign'], 'Orientation');
      |       delete_block([gcb '/f32IQErrSign']);
      |       add_block('built-in/Outport', [gcb '/f32IQErrSign'], 'Position', pos, 'Orientation', orient);
      | 
      |       pos = get_param([gcb '/f32IQErr'], 'Position');
      |       orient = get_param([gcb '/f32IQErr'], 'Orientation');
      |       delete_block([gcb '/f32IQErr']);
      |       add_block('built-in/Outport', [gcb '/f32IQErr'], 'Position', pos, 'Orientation', orient);
      | 
      |       pos = get_param([gcb '/f32FWErr'], 'Position');
      |       orient = get_param([gcb '/f32FWErr'], 'Orientation');
      |       delete_block([gcb '/f32FWErr']);
      |       add_block('built-in/Outport', [gcb '/f32FWErr'], 'Position', pos, 'Orientation', orient);
      | 
      |       pos = get_param([gcb '/f32UQErr'], 'Position');
      |       orient = get_param([gcb '/f32UQErr'], 'Orientation');
      |       delete_block([gcb '/f32UQErr']);
      |       add_block('built-in/Outport', [gcb '/f32UQErr'], 'Position', pos, 'Orientation', orient);
      | 
      |       pos = get_param([gcb '/f32FWErrFilt'], 'Position');
      |       orient = get_param([gcb '/f32FWErrFilt'], 'Orientation');
      |       delete_block([gcb '/f32FWErrFilt']);
      |       add_block('built-in/Outport', [gcb '/f32FWErrFilt'], 'Position', pos, 'Orientation', orient);
      | 
      |       pos = get_param([gcb '/f32FWAngle'], 'Position');
      |       orient = get_param([gcb '/f32FWAngle'], 'Orientation');
      |       delete_block([gcb '/f32FWAngle']);
      |       add_block('built-in/Outport', [gcb '/f32FWAngle'], 'Position', pos, 'Orientation', orient);
      | 
      |       pos = get_param([gcb '/f32FWSin'], 'Position');
      |       orient = get_param([gcb '/f32FWSin'], 'Orientation');
      |       delete_block([gcb '/f32FWSin']);
      |       add_block('built-in/Outport', [gcb '/f32FWSin'], 'Position', pos, 'Orientation', orient);
      | 
      |       pos = get_param([gcb '/f32FWCos'], 'Position');
      |       orient = get_param([gcb '/f32FWCos'], 'Orientation');
      |       delete_block([gcb '/f32FWCos']);
      |       add_block('built-in/Outport', [gcb '/f32FWCos'], 'Position', pos, 'Orientation', orient);
      | 
      |       tmpOutCnt=0;
      |       tmpOutCnt=tmpOutCnt+1;
      |       set_param([gcb '/pIDQReq'], 'Port', num2str(tmpOutCnt));
      |       tmpOutCnt=tmpOutCnt+1;
      |       set_param([gcb '/u16LimitFlagQ'], 'Port', num2str(tmpOutCnt));
      |       tmpOutCnt=tmpOutCnt+1;
      |       set_param([gcb '/u16LimitFlagFW'], 'Port', num2str(tmpOutCnt));
      |       tmpOutCnt=tmpOutCnt+1;
      |       set_param([gcb '/f32WReqFilt'], 'Port', num2str(tmpOutCnt));
      |       tmpOutCnt=tmpOutCnt+1;
      |       set_param([gcb '/f32WErr'], 'Port', num2str(tmpOutCnt));
      |       tmpOutCnt=tmpOutCnt+1;
      |       set_param([gcb '/f32WFbckFilt'], 'Port', num2str(tmpOutCnt));
      |       tmpOutCnt=tmpOutCnt+1;
      |       set_param([gcb '/f32IDQReqAmp'], 'Port', num2str(tmpOutCnt));
      |       tmpOutCnt=tmpOutCnt+1;
      |       set_param([gcb '/f32IQErrSign'], 'Port', num2str(tmpOutCnt));
      |       tmpOutCnt=tmpOutCnt+1;
      |       set_param([gcb '/f32IQErr'], 'Port', num2str(tmpOutCnt));
      |       tmpOutCnt=tmpOutCnt+1;
      |       set_param([gcb '/f32FWErr'], 'Port', num2str(tmpOutCnt));
      |       tmpOutCnt=tmpOutCnt+1;
      |       set_param([gcb '/f32UQErr'], 'Port', num2str(tmpOutCnt));
      |       tmpOutCnt=tmpOutCnt+1;
      |       set_param([gcb '/f32FWErrFilt'], 'Port', num2str(tmpOutCnt));
      |       tmpOutCnt=tmpOutCnt+1;
      |       set_param([gcb '/f32FWAngle'], 'Port', num2str(tmpOutCnt));
      |       tmpOutCnt=tmpOutCnt+1;
      |       set_param([gcb '/f32FWSin'], 'Port', num2str(tmpOutCnt));
      |       tmpOutCnt=tmpOutCnt+1;
      |       set_param([gcb '/f32FWCos'], 'Port', num2str(tmpOutCnt));
      |       tmpOutCnt=tmpOutCnt+1;
      |       set_param([gcb '/f32AccW_Out'], 'Port', num2str(tmpOutCnt));
      |       tmpOutCnt=tmpOutCnt+1;
      |       set_param([gcb '/f32AccFW_Out'], 'Port', num2str(tmpOutCnt));
      |       tmpOutCnt=tmpOutCnt+1;
      |       set_param([gcb '/f32IntegPartK_1Q_Out'], 'Port', num2str(tmpOutCnt));
      |       tmpOutCnt=tmpOutCnt+1;
      |       set_param([gcb '/f32InK_1Q_Out'], 'Port', num2str(tmpOutCnt));
      |       tmpOutCnt=tmpOutCnt+1;
      |       set_param([gcb '/f32IntegPartK_1FW_Out'], 'Port', num2str(tmpOutCnt));
      |       tmpOutCnt=tmpOutCnt+1;
      |       set_param([gcb '/f32InK_1FW_Out'], 'Port', num2str(tmpOutCnt));
      |       if strcmp(get_param([gcb '/f32State_Out'], 'BlockType'), 'Outport')
      |         tmpOutCnt=tmpOutCnt+1;
      |         set_param([gcb '/f32State_Out'], 'Port', num2str(tmpOutCnt));
      |       end
      |     elseif (showDebugOutputs == 1) && (strcmp(get_param([gcb '/f32WReqFilt'], 'BlockType'), 'Outport'))
      |       % hidden debugging outputs
      |       pos = get_param([gcb '/f32WReqFilt'], 'Position');
      |       orient = get_param([gcb '/f32WReqFilt'], 'Orientation');
      |       delete_block([gcb '/f32WReqFilt']);
      |       add_block('built-in/Terminator', [gcb '/f32WReqFilt'], 'Position', pos, 'Orientation', orient);
      | 
      |       pos = get_param([gcb '/f32WErr'], 'Position');
      |       orient = get_param([gcb '/f32WErr'], 'Orientation');
      |       delete_block([gcb '/f32WErr']);
      |       add_block('built-in/Terminator', [gcb '/f32WErr'], 'Position', pos, 'Orientation', orient);
      | 
      |       pos = get_param([gcb '/f32WFbckFilt'], 'Position');
      |       orient = get_param([gcb '/f32WFbckFilt'], 'Orientation');
      |       delete_block([gcb '/f32WFbckFilt']);
      |       add_block('built-in/Terminator', [gcb '/f32WFbckFilt'], 'Position', pos, 'Orientation', orient);
      | 
      |       pos = get_param([gcb '/f32IDQReqAmp'], 'Position');
      |       orient = get_param([gcb '/f32IDQReqAmp'], 'Orientation');
      |       delete_block([gcb '/f32IDQReqAmp']);
      |       add_block('built-in/Terminator', [gcb '/f32IDQReqAmp'], 'Position', pos, 'Orientation', orient);
      | 
      |       pos = get_param([gcb '/f32IQErrSign'], 'Position');
      |       orient = get_param([gcb '/f32IQErrSign'], 'Orientation');
      |       delete_block([gcb '/f32IQErrSign']);
      |       add_block('built-in/Terminator', [gcb '/f32IQErrSign'], 'Position', pos, 'Orientation', orient);
      | 
      |       pos = get_param([gcb '/f32IQErr'], 'Position');
      |       orient = get_param([gcb '/f32IQErr'], 'Orientation');
      |       delete_block([gcb '/f32IQErr']);
      |       add_block('built-in/Terminator', [gcb '/f32IQErr'], 'Position', pos, 'Orientation', orient);
      | 
      |       pos = get_param([gcb '/f32FWErr'], 'Position');
      |       orient = get_param([gcb '/f32FWErr'], 'Orientation');
      |       delete_block([gcb '/f32FWErr']);
      |       add_block('built-in/Terminator', [gcb '/f32FWErr'], 'Position', pos, 'Orientation', orient);
      | 
      |       pos = get_param([gcb '/f32UQErr'], 'Position');
      |       orient = get_param([gcb '/f32UQErr'], 'Orientation');
      |       delete_block([gcb '/f32UQErr']);
      |       add_block('built-in/Terminator', [gcb '/f32UQErr'], 'Position', pos, 'Orientation', orient);
      | 
      |       pos = get_param([gcb '/f32FWErrFilt'], 'Position');
      |       orient = get_param([gcb '/f32FWErrFilt'], 'Orientation');
      |       delete_block([gcb '/f32FWErrFilt']);
      |       add_block('built-in/Terminator', [gcb '/f32FWErrFilt'], 'Position', pos, 'Orientation', orient);
      | 
      |       pos = get_param([gcb '/f32FWAngle'], 'Position');
      |       orient = get_param([gcb '/f32FWAngle'], 'Orientation');
      |       delete_block([gcb '/f32FWAngle']);
      |       add_block('built-in/Terminator', [gcb '/f32FWAngle'], 'Position', pos, 'Orientation', orient);
      | 
      |       pos = get_param([gcb '/f32FWSin'], 'Position');
      |       orient = get_param([gcb '/f32FWSin'], 'Orientation');
      |       delete_block([gcb '/f32FWSin']);
      |       add_block('built-in/Terminator', [gcb '/f32FWSin'], 'Position', pos, 'Orientation', orient);
      | 
      |       pos = get_param([gcb '/f32FWCos'], 'Position');
      |       orient = get_param([gcb '/f32FWCos'], 'Orientation');
      |       delete_block([gcb '/f32FWCos']);
      |       add_block('built-in/Terminator', [gcb '/f32FWCos'], 'Position', pos, 'Orientation', orient);
      | 
      |       tmpOutCnt=0;
      |       tmpOutCnt=tmpOutCnt+1;
      |       set_param([gcb '/pIDQReq'], 'Port', num2str(tmpOutCnt));
      |       tmpOutCnt=tmpOutCnt+1;
      |       set_param([gcb '/u16LimitFlagQ'], 'Port', num2str(tmpOutCnt));
      |       tmpOutCnt=tmpOutCnt+1;
      |       set_param([gcb '/u16LimitFlagFW'], 'Port', num2str(tmpOutCnt));
      |       tmpOutCnt=tmpOutCnt+1;
      |       set_param([gcb '/f32AccW_Out'], 'Port', num2str(tmpOutCnt));
      |       tmpOutCnt=tmpOutCnt+1;
      |       set_param([gcb '/f32AccFW_Out'], 'Port', num2str(tmpOutCnt));
      |       tmpOutCnt=tmpOutCnt+1;
      |       set_param([gcb '/f32IntegPartK_1Q_Out'], 'Port', num2str(tmpOutCnt));
      |       tmpOutCnt=tmpOutCnt+1;
      |       set_param([gcb '/f32InK_1Q_Out'], 'Port', num2str(tmpOutCnt));
      |       tmpOutCnt=tmpOutCnt+1;
      |       set_param([gcb '/f32IntegPartK_1FW_Out'], 'Port', num2str(tmpOutCnt));
      |       tmpOutCnt=tmpOutCnt+1;
      |       set_param([gcb '/f32InK_1FW_Out'], 'Port', num2str(tmpOutCnt));
      |       if strcmp(get_param([gcb '/f32State_Out'], 'BlockType'), 'Outport')
      |         tmpOutCnt=tmpOutCnt+1;
      |         set_param([gcb '/f32State_Out'], 'Port', num2str(tmpOutCnt));
      |       end
      |     end
      |   end
      | end
      | if strcmp(get_param(gcb,'f32State_Out_showOutput'),'on')
      |   if strcmp(get_param([gcb '/f32State_Out'], 'BlockType'), 'Terminator')
      |     pos = get_param([gcb '/f32State_Out'], 'Position');
      |     orient = get_param([gcb '/f32State_Out'], 'Orientation');
      |     delete_block([gcb '/f32State_Out']);
      |     add_block('built-in/Outport', [gcb '/f32State_Out'], 'Position', pos, 'Orientation', orient);
      |     outputsChanged = 1;
      |   end
      | else
      |   if strcmp(get_param([gcb '/f32State_Out'], 'BlockType'), 'Outport')
      |     pos = get_param([gcb '/f32State_Out'], 'Position');
      |     orient = get_param([gcb '/f32State_Out'], 'Orientation');
      |     delete_block([gcb '/f32State_Out']);
      |     add_block('built-in/Terminator', [gcb '/f32State_Out'], 'Position', pos, 'Orientation', orient);
      |     outputsChanged = 1;
      |   end
      | end
      | if outputsChanged == 1;
      |   tmpOutCnt = 0;
      |   if strcmp(get_param([gcb '/pIDQReq'], 'BlockType'), 'Outport')
      |     tmpOutCnt = tmpOutCnt + 1;
      |     set_param([gcb '/pIDQReq'], 'Port', num2str(tmpOutCnt));
      |   end
      |   if strcmp(get_param([gcb '/u16LimitFlagQ'], 'BlockType'), 'Outport')
      |     tmpOutCnt = tmpOutCnt + 1;
      |     set_param([gcb '/u16LimitFlagQ'], 'Port', num2str(tmpOutCnt));
      |   end
      |   if strcmp(get_param([gcb '/u16LimitFlagFW'], 'BlockType'), 'Outport')
      |     tmpOutCnt = tmpOutCnt + 1;
      |     set_param([gcb '/u16LimitFlagFW'], 'Port', num2str(tmpOutCnt));
      |   end
      |   if strcmp(get_param([gcb '/f32WReqFilt'], 'BlockType'), 'Outport')
      |     tmpOutCnt = tmpOutCnt + 1;
      |     set_param([gcb '/f32WReqFilt'], 'Port', num2str(tmpOutCnt));
      |   end
      |   if strcmp(get_param([gcb '/f32WErr'], 'BlockType'), 'Outport')
      |     tmpOutCnt = tmpOutCnt + 1;
      |     set_param([gcb '/f32WErr'], 'Port', num2str(tmpOutCnt));
      |   end
      |   if strcmp(get_param([gcb '/f32WFbckFilt'], 'BlockType'), 'Outport')
      |     tmpOutCnt = tmpOutCnt + 1;
      |     set_param([gcb '/f32WFbckFilt'], 'Port', num2str(tmpOutCnt));
      |   end
      |   if strcmp(get_param([gcb '/f32IDQReqAmp'], 'BlockType'), 'Outport')
      |     tmpOutCnt = tmpOutCnt + 1;
      |     set_param([gcb '/f32IDQReqAmp'], 'Port', num2str(tmpOutCnt));
      |   end
      |   if strcmp(get_param([gcb '/f32IQErrSign'], 'BlockType'), 'Outport')
      |     tmpOutCnt = tmpOutCnt + 1;
      |     set_param([gcb '/f32IQErrSign'], 'Port', num2str(tmpOutCnt));
      |   end
      |   if strcmp(get_param([gcb '/f32IQErr'], 'BlockType'), 'Outport')
      |     tmpOutCnt = tmpOutCnt + 1;
      |     set_param([gcb '/f32IQErr'], 'Port', num2str(tmpOutCnt));
      |   end
      |   if strcmp(get_param([gcb '/f32FWErr'], 'BlockType'), 'Outport')
      |     tmpOutCnt = tmpOutCnt + 1;
      |     set_param([gcb '/f32FWErr'], 'Port', num2str(tmpOutCnt));
      |   end
      |   if strcmp(get_param([gcb '/f32UQErr'], 'BlockType'), 'Outport')
      |     tmpOutCnt = tmpOutCnt + 1;
      |     set_param([gcb '/f32UQErr'], 'Port', num2str(tmpOutCnt));
      |   end
      |   if strcmp(get_param([gcb '/f32FWErrFilt'], 'BlockType'), 'Outport')
      |     tmpOutCnt = tmpOutCnt + 1;
      |     set_param([gcb '/f32FWErrFilt'], 'Port', num2str(tmpOutCnt));
      |   end
      |   if strcmp(get_param([gcb '/f32FWAngle'], 'BlockType'), 'Outport')
      |     tmpOutCnt = tmpOutCnt + 1;
      |     set_param([gcb '/f32FWAngle'], 'Port', num2str(tmpOutCnt));
      |   end
      |   if strcmp(get_param([gcb '/f32FWSin'], 'BlockType'), 'Outport')
      |     tmpOutCnt = tmpOutCnt + 1;
      |     set_param([gcb '/f32FWSin'], 'Port', num2str(tmpOutCnt));
      |   end
      |   if strcmp(get_param([gcb '/f32FWCos'], 'BlockType'), 'Outport')
      |     tmpOutCnt = tmpOutCnt + 1;
      |     set_param([gcb '/f32FWCos'], 'Port', num2str(tmpOutCnt));
      |   end
      |   if strcmp(get_param([gcb '/f32AccW_Out'], 'BlockType'), 'Outport')
      |     tmpOutCnt = tmpOutCnt + 1;
      |     set_param([gcb '/f32AccW_Out'], 'Port', num2str(tmpOutCnt));
      |   end
      |   if strcmp(get_param([gcb '/f32AccFW_Out'], 'BlockType'), 'Outport')
      |     tmpOutCnt = tmpOutCnt + 1;
      |     set_param([gcb '/f32AccFW_Out'], 'Port', num2str(tmpOutCnt));
      |   end
      |   if strcmp(get_param([gcb '/f32IntegPartK_1Q_Out'], 'BlockType'), 'Outport')
      |     tmpOutCnt = tmpOutCnt + 1;
      |     set_param([gcb '/f32IntegPartK_1Q_Out'], 'Port', num2str(tmpOutCnt));
      |   end
      |   if strcmp(get_param([gcb '/f32InK_1Q_Out'], 'BlockType'), 'Outport')
      |     tmpOutCnt = tmpOutCnt + 1;
      |     set_param([gcb '/f32InK_1Q_Out'], 'Port', num2str(tmpOutCnt));
      |   end
      |   if strcmp(get_param([gcb '/f32IntegPartK_1FW_Out'], 'BlockType'), 'Outport')
      |     tmpOutCnt = tmpOutCnt + 1;
      |     set_param([gcb '/f32IntegPartK_1FW_Out'], 'Port', num2str(tmpOutCnt));
      |   end
      |   if strcmp(get_param([gcb '/f32InK_1FW_Out'], 'BlockType'), 'Outport')
      |     tmpOutCnt = tmpOutCnt + 1;
      |     set_param([gcb '/f32InK_1FW_Out'], 'Port', num2str(tmpOutCnt));
      |   end
      |   if strcmp(get_param([gcb '/f32State_Out'], 'BlockType'), 'Outport')
      |     tmpOutCnt = tmpOutCnt + 1;
      |     set_param([gcb '/f32State_Out'], 'Port', num2str(tmpOutCnt));
      |   end
      | end
      settings: RTWSystemCode=Inline
      mask Help: web([fileparts(which('ammclib_bam_S32K3xx.slx')) '/../doc/S32K3XXMCLUG.pdf'], '-browser')
      mask TypeOptions showStates: Hide (faster execution) | Show (allows debugging; connect feedback loops manually)
      mask Callback showStates:
      | maskStr=get_param(gcb,'showStates');
      | if strcmp(maskStr,'Hide (faster execution)')
      |   autoCalcEn=get_param(gcb,'autoCalcEn');
      |   if strcmp(autoCalcEn,'on')
      |     set_param(gcb,'MaskEnables',{'on','on','off','on','on','on','on','on','on','on','on','on','on','on','on','on','on','on','on','on','on','on','on','on','on','on','on','on','on','on','on','on','on','on','off'});
      |   else
      |     set_param(gcb,'MaskEnables',{'on','on','off','on','on','off','off','off','off','off','off','off','off','off','off','off','off','on','on','on','on','on','on','on','on','on','on','on','on','on','on','on','on','on','off'});
      |   end
      | else
      |   set_param(gcb,'MaskEnables',{'on','on','on','on','on','off','off','off','off','off','off','off','off','off','off','off','off','off','off','off','off','off','off','off','off','off','off','off','off','off','off','off','off','off','off'});
      | end
      mask TypeOptions resetStatesEnable: Pre-set according to the first set of inputs after reset | Clear to zero
      mask TypeOptions showDebugOutputs: Hide | Show
      mask TypeOptions SampleTime: f32VelocityReq/SampleTime | f32VelocityFbck/SampleTime | f32IQFbck/SampleTime | f32UQReq/SampleTime | f32UQLim/SampleTime | f32FilterMAWOut_preset/SampleTime | f32FilterMAFWOut_preset/SampleTime | f32ControllerPIpAWQOut_preset/SampleTime | f32ControllerPIpAWFWOut_preset/SampleTime | f32RampOut_preset/SampleTime
      mask Callback SampleTime:
      | p=Simulink.Mask.get(gcb);
      | hintText=p.getDialogControl('timeHint');
      | SampleTime=Simulink.data.evalinGlobal(bdroot,get_param(gcb,'SampleTime'));
      | SampleTime_1=str2double(get_param(gcb,'SampleTime_1'));
      | if (((SampleTime==-1) && (~contains(hintText.Prompt,'inherited'))) || ...
      |     ((SampleTime~=-1) && contains(hintText.Prompt,'inherited')) || ...
      |     ((SampleTime~=-1) && (SampleTime_1~=SampleTime)) || ...
      |     ((SampleTime_1~=-1) && contains(hintText.Prompt,'yet')))
      |   if ((SampleTime==-1) && (~contains(hintText.Prompt,'inherited')))
      |     set_param(gcb,'SampleTime_1',num2str(NaN));
      |     SampleTime_1=NaN;
      |   end
      |   if (SampleTime~=-1)
      |     set_param(gcb,'SampleTime_1',num2str(SampleTime));
      |     SampleTime_1=SampleTime;
      |   end
      |   autoCalcEn=get_param(gcb,'autoCalcEn');
      |   if strcmp(autoCalcEn,'on')
      |     p=Simulink.Mask.get(gcb);
      |     hintText=p.getDialogControl('timeHint');
      |     if SampleTime==-1
      |       SampleTime=SampleTime_1;
      |       if isnan(SampleTime)
      |         hintText.Prompt='Note: Implementation parameters cannot be calculated yet because the block''s inherited sample time is unknown. Simulink will update the sample time when you run the simulation.';
      |       else
      |         hintText.Prompt='Caution: Implementation parameters depend on inherited sample time. Make sure that the sample time of the block''s inputs corresponds to the sampling period in the target application.';
      |       end
      |     else
      |       hintText.Prompt='Caution: Implementation parameters depend on the sample time. Make sure that the simulation time step corresponds to the sampling period in the target application.';
      |     end
      |     u16NSamplesW_bkup=get_param(gcb,'u16NSamplesW');
      |     u16NSamplesFW_bkup=get_param(gcb,'u16NSamplesFW');
      |     f32PropGainQ_bkup=get_param(gcb,'f32PropGainQ');
      |     f32IntegGainQ_bkup=get_param(gcb,'f32IntegGainQ');
      |     s16PropGainShiftQ_bkup=get_param(gcb,'s16PropGainShiftQ');
      |     s16IntegGainShiftQ_bkup=get_param(gcb,'s16IntegGainShiftQ');
      |     f32LowerLimitQ_bkup=get_param(gcb,'f32LowerLimitQ');
      |     f32UpperLimitQ_bkup=get_param(gcb,'f32UpperLimitQ');
      |     f32PropGainFW_bkup=get_param(gcb,'f32PropGainFW');
      |     f32IntegGainFW_bkup=get_param(gcb,'f32IntegGainFW');
      |     s16PropGainShiftFW_bkup=get_param(gcb,'s16PropGainShiftFW');
      |     s16IntegGainShiftFW_bkup=get_param(gcb,'s16IntegGainShiftFW');
      |     f32LowerLimitFW_bkup=get_param(gcb,'f32LowerLimitFW');
      |     f32UpperLimitFW_bkup=get_param(gcb,'f32UpperLimitFW');
      |     f32RampUp_bkup=get_param(gcb,'f32RampUp');
      |     f32RampDown_bkup=get_param(gcb,'f32RampDown');
      |     wf0=Simulink.data.evalinGlobal(bdroot,get_param(gcb,'wf0'));
      |     wksi=Simulink.data.evalinGlobal(bdroot,get_param(gcb,'wksi'));
      |     J=Simulink.data.evalinGlobal(bdroot,get_param(gcb,'J'));
      |     Kt=Simulink.data.evalinGlobal(bdroot,get_param(gcb,'Kt'));
      |     lambdaW=Simulink.data.evalinGlobal(bdroot,get_param(gcb,'lambdaW'));
      |     lambdaFW=Simulink.data.evalinGlobal(bdroot,get_param(gcb,'lambdaFW'));
      |     Idmax=Simulink.data.evalinGlobal(bdroot,get_param(gcb,'Idmax'));
      |     ramprpm=Simulink.data.evalinGlobal(bdroot,get_param(gcb,'ramprpm'));
      |     mechspeed=Simulink.data.evalinGlobal(bdroot,get_param(gcb,'mechspeed'));
      |     polepairs=Simulink.data.evalinGlobal(bdroot,get_param(gcb,'polepairs'));
      |     uscale=Simulink.data.evalinGlobal(bdroot,get_param(gcb,'uscale'));
      |     iscale=Simulink.data.evalinGlobal(bdroot,get_param(gcb,'iscale'));
      |     if (wf0<=0)
      |       warning('Natural frequency f0 must be positive.');
      |     end
      |     if (wksi<=0)
      |       warning('Current loop attenuation must be positive.');
      |     end
      |     if (wksi>1)
      |       warning('Current loop attenuation must not exceed 1.');
      |     end
      |     if (J<=0)
      |       warning('Moment of inertia J must be positive.');
      |     end
      |     if (Kt<=0)
      |       warning('Torque constant Kt must be positive.');
      |     end
      |     if (lambdaW<0)
      |       warning('MA filter smoothing factor must be in the range 0..1.');
      |     end
      |     if (lambdaW>1)
      |       warning('MA filter smoothing factor must be in the range 0..1.');
      |     end
      |     if (lambdaFW<0)
      |       warning('MA filter smoothing factor must be in the range 0..1.');
      |     end
      |     if (lambdaFW>1)
      |       warning('MA filter smoothing factor must be in the range 0..1.');
      |     end
      |     if (mechspeed<=0)
      |       warning('Max. speed must be positive.');
      |     end
      |     if (polepairs<1)
      |       warning('Number of pole pairs must be a natural number (1, 2, 3, ...).');
      |     end
      |     if (round(polepairs)~=polepairs)
      |       warning('Number of pole pairs must be a natural number (1, 2, 3, ...).');
      |     end
      |     if (uscale<=0)
      |       warning('U_max must be positive.');
      |     end
      |     if (iscale<=0)
      |       warning('I_max must be positive.');
      |     end
      |     w0=6.283185307179586*wf0;
      |     pgain=2.0*wksi*w0*J/Kt;
      |     igain=w0*w0*J/Kt;
      |     wmax=polepairs*mechspeed*0.1047197551196598;
      |     kpf=pgain*wmax/iscale;
      |     s16PropGainShiftQ=ceil(log2(abs(kpf)));
      |     if s16PropGainShiftQ<-31
      |       s16PropGainShiftQ=-31;
      |     end
      |     if s16PropGainShiftQ>31
      |       s16PropGainShiftQ=31;
      |       warning(['Parameter s16PropGainShiftQ of ' gcb ' exceeds the fixed-point range.']);
      |     end
      |     f32PropGainQ=round(kpf*2^(-s16PropGainShiftQ)*2^31);
      |     if f32PropGainQ>2^31-1
      |       f32PropGainQ=2^31-1;
      |       warning(['Parameter f32PropGainQ of ' gcb ' exceeds the fixed-point range.']);
      |     end
      |     if f32PropGainQ<-2^31
      |       f32PropGainQ=-2^31;
      |       warning(['Parameter f32PropGainQ of ' gcb ' exceeds the fixed-point range.']);
      |     end
      |     kif=igain*SampleTime*0.5*wmax/iscale;
      |     s16IntegGainShiftQ=ceil(log2(abs(kif)));
      |     if s16IntegGainShiftQ<-31
      |       s16IntegGainShiftQ=-31;
      |     end
      |     if s16IntegGainShiftQ>31
      |       s16IntegGainShiftQ=31;
      |       warning(['Parameter s16IntegGainShiftQ of ' gcb ' exceeds the fixed-point range.']);
      |     end
      |     f32IntegGainQ=round(kif*2^(-s16IntegGainShiftQ)*2^31);
      |     if f32IntegGainQ>2^31-1
      |       f32IntegGainQ=2^31-1;
      |       warning(['Parameter f32IntegGainQ of ' gcb ' exceeds the fixed-point range.']);
      |     end
      |     if f32IntegGainQ<-2^31
      |       f32IntegGainQ=-2^31;
      |       warning(['Parameter f32IntegGainQ of ' gcb ' exceeds the fixed-point range.']);
      |     end
      |     f32LowerLimitQ=-2147483648;
      |     f32UpperLimitQ=2147483647;
      |     fwkpf=0.9*pgain*wmax/iscale;
      |     s16PropGainShiftFW=ceil(log2(abs(fwkpf)));
      |     if s16PropGainShiftFW<-31
      |       s16PropGainShiftFW=-31;
      |     end
      |     if s16PropGainShiftFW>31
      |       s16PropGainShiftFW=31;
      |       warning(['Parameter s16PropGainShiftFW of ' gcb ' exceeds the fixed-point range.']);
      |     end
      |     f32PropGainFW=round(fwkpf*2^(-s16PropGainShiftFW)*2^31);
      |     if f32PropGainFW>2^31-1
      |       f32PropGainFW=2^31-1;
      |       warning(['Parameter f32PropGainFW of ' gcb ' exceeds the fixed-point range.']);
      |     end
      |     if f32PropGainFW<-2^31
      |       f32PropGainFW=-2^31;
      |       warning(['Parameter f32PropGainFW of ' gcb ' exceeds the fixed-point range.']);
      |     end
      |     s16IntegGainShiftFW=s16IntegGainShiftQ;
      |     f32IntegGainFW=f32IntegGainQ;
      |     if (Idmax<0)
      |       iratio=abs(Idmax)/iscale;
      |       if (abs(iratio) > 1)
      |         iratio = 0;
      |       end
      |       lowlim=0.3183098861837907*acos(iratio)-0.5;
      |     else
      |       lowlim=0.0;
      |     end
      |     f32LowerLimitFW=round(lowlim*2^31);
      |     if f32LowerLimitFW>2^31-1
      |       f32LowerLimitFW=2^31-1;
      |       warning(['Parameter f32LowerLimitFW of ' gcb ' exceeds the fixed-point range.']);
      |     end
      |     if f32LowerLimitFW<-2^31
      |       f32LowerLimitFW=-2^31;
      |       warning(['Parameter f32LowerLimitFW of ' gcb ' exceeds the fixed-point range.']);
      |     end
      |     f32UpperLimitFW=0;
      |     u16NSamplesW=round(log2(1.0/abs(lambdaW)));
      |     if u16NSamplesW>31
      |       u16NSamplesW=31;
      |     end
      |     if u16NSamplesW<0
      |       u16NSamplesW=0;
      |     end
      |     u16NSamplesFW=round(log2(1.0/abs(lambdaFW)));
      |     if u16NSamplesFW>31
      |       u16NSamplesFW=31;
      |     end
      |     if u16NSamplesFW<0
      |       u16NSamplesFW=0;
      |     end
      |     rampsc=polepairs*abs(ramprpm)*0.1047197551196598/wmax;
      |     f32RampUp=round(rampsc*2^31);
      |     if f32RampUp>2^31-1
      |       f32RampUp=2^31-1;
      |       warning(['Parameter f32RampUp of ' gcb ' exceeds the fixed-point range.']);
      |     end
      |     if f32RampUp<-2^31
      |       f32RampUp=-2^31;
      |       warning(['Parameter f32RampUp of ' gcb ' exceeds the fixed-point range.']);
      |     end
      |     f32RampDown=round(rampsc*2^31);
      |     if f32RampDown>2^31-1
      |       f32RampDown=2^31-1;
      |       warning(['Parameter f32RampDown of ' gcb ' exceeds the fixed-point range.']);
      |     end
      |     if f32RampDown<-2^31
      |       f32RampDown=-2^31;
      |       warning(['Parameter f32RampDown of ' gcb ' exceeds the fixed-point range.']);
      |     end
      |     if isnan(u16NSamplesW)
      |       if ~strcmp(u16NSamplesW_bkup,'0')
      |         set_param(gcb,'u16NSamplesW','0');
      |       end
      |     else
      |       tmps=num2str(u16NSamplesW);
      |       if ~strcmp(u16NSamplesW_bkup,tmps)
      |         set_param(gcb,'u16NSamplesW',tmps);
      |       end
      |     end
      |     if isnan(u16NSamplesFW)
      |       if ~strcmp(u16NSamplesFW_bkup,'0')
      |         set_param(gcb,'u16NSamplesFW','0');
      |       end
      |     else
      |       tmps=num2str(u16NSamplesFW);
      |       if ~strcmp(u16NSamplesFW_bkup,tmps)
      |         set_param(gcb,'u16NSamplesFW',tmps);
      |       end
      |     end
      |     if isnan(f32PropGainQ)
      |       if ~strcmp(f32PropGainQ_bkup,'0')
      |         set_param(gcb,'f32PropGainQ','0');
      |       end
      |     else
      |       tmps=num2str(f32PropGainQ);
      |       if ~strcmp(f32PropGainQ_bkup,tmps)
      |         set_param(gcb,'f32PropGainQ',tmps);
      |       end
      |     end
      |     if isnan(f32IntegGainQ)
      |       if ~strcmp(f32IntegGainQ_bkup,'0')
      |         set_param(gcb,'f32IntegGainQ','0');
      |       end
      |     else
      |       tmps=num2str(f32IntegGainQ);
      |       if ~strcmp(f32IntegGainQ_bkup,tmps)
      |         set_param(gcb,'f32IntegGainQ',tmps);
      |       end
      |     end
      |     if isnan(s16PropGainShiftQ)
      |       if ~strcmp(s16PropGainShiftQ_bkup,'0')
      |         set_param(gcb,'s16PropGainShiftQ','0');
      |       end
      |     else
      |       tmps=num2str(s16PropGainShiftQ);
      |       if ~strcmp(s16PropGainShiftQ_bkup,tmps)
      |         set_param(gcb,'s16PropGainShiftQ',tmps);
      |       end
      |     end
      |     if isnan(s16IntegGainShiftQ)
      |       if ~strcmp(s16IntegGainShiftQ_bkup,'0')
      |         set_param(gcb,'s16IntegGainShiftQ','0');
      |       end
      |     else
      |       tmps=num2str(s16IntegGainShiftQ);
      |       if ~strcmp(s16IntegGainShiftQ_bkup,tmps)
      |         set_param(gcb,'s16IntegGainShiftQ',tmps);
      |       end
      |     end
      |     if isnan(f32LowerLimitQ)
      |       if ~strcmp(f32LowerLimitQ_bkup,'0')
      |         set_param(gcb,'f32LowerLimitQ','0');
      |       end
      |     else
      |       tmps=num2str(f32LowerLimitQ);
      |       if ~strcmp(f32LowerLimitQ_bkup,tmps)
      |         set_param(gcb,'f32LowerLimitQ',tmps);
      |       end
      |     end
      |     if isnan(f32UpperLimitQ)
      |       if ~strcmp(f32UpperLimitQ_bkup,'0')
      |         set_param(gcb,'f32UpperLimitQ','0');
      |       end
      |     else
      |       tmps=num2str(f32UpperLimitQ);
      |       if ~strcmp(f32UpperLimitQ_bkup,tmps)
      |         set_param(gcb,'f32UpperLimitQ',tmps);
      |       end
      |     end
      |     if isnan(f32PropGainFW)
      |       if ~strcmp(f32PropGainFW_bkup,'0')
      |         set_param(gcb,'f32PropGainFW','0');
      |       end
      |     else
      |       tmps=num2str(f32PropGainFW);
      |       if ~strcmp(f32PropGainFW_bkup,tmps)
      |         set_param(gcb,'f32PropGainFW',tmps);
      |       end
      |     end
      |     if isnan(f32IntegGainFW)
      |       if ~strcmp(f32IntegGainFW_bkup,'0')
      |         set_param(gcb,'f32IntegGainFW','0');
      |       end
      |     else
      |       tmps=num2str(f32IntegGainFW);
      |       if ~strcmp(f32IntegGainFW_bkup,tmps)
      |         set_param(gcb,'f32IntegGainFW',tmps);
      |       end
      |     end
      |     if isnan(s16PropGainShiftFW)
      |       if ~strcmp(s16PropGainShiftFW_bkup,'0')
      |         set_param(gcb,'s16PropGainShiftFW','0');
      |       end
      |     else
      |       tmps=num2str(s16PropGainShiftFW);
      |       if ~strcmp(s16PropGainShiftFW_bkup,tmps)
      |         set_param(gcb,'s16PropGainShiftFW',tmps);
      |       end
      |     end
      |     if isnan(s16IntegGainShiftFW)
      |       if ~strcmp(s16IntegGainShiftFW_bkup,'0')
      |         set_param(gcb,'s16IntegGainShiftFW','0');
      |       end
      |     else
      |       tmps=num2str(s16IntegGainShiftFW);
      |       if ~strcmp(s16IntegGainShiftFW_bkup,tmps)
      |         set_param(gcb,'s16IntegGainShiftFW',tmps);
      |       end
      |     end
      |     if isnan(f32LowerLimitFW)
      |       if ~strcmp(f32LowerLimitFW_bkup,'0')
      |         set_param(gcb,'f32LowerLimitFW','0');
      |       end
      |     else
      |       tmps=num2str(f32LowerLimitFW);
      |       if ~strcmp(f32LowerLimitFW_bkup,tmps)
      |         set_param(gcb,'f32LowerLimitFW',tmps);
      |       end
      |     end
      |     if isnan(f32UpperLimitFW)
      |       if ~strcmp(f32UpperLimitFW_bkup,'0')
      |         set_param(gcb,'f32UpperLimitFW','0');
      |       end
      |     else
      |       tmps=num2str(f32UpperLimitFW);
      |       if ~strcmp(f32UpperLimitFW_bkup,tmps)
      |         set_param(gcb,'f32UpperLimitFW',tmps);
      |       end
      |     end
      |     if isnan(f32RampUp)
      |       if ~strcmp(f32RampUp_bkup,'0')
      |         set_param(gcb,'f32RampUp','0');
      |       end
      |     else
      |       tmps=num2str(f32RampUp);
      |       if ~strcmp(f32RampUp_bkup,tmps)
      |         set_param(gcb,'f32RampUp',tmps);
      |       end
      |     end
      |     if isnan(f32RampDown)
      |       if ~strcmp(f32RampDown_bkup,'0')
      |         set_param(gcb,'f32RampDown','0');
      |       end
      |     else
      |       tmps=num2str(f32RampDown);
      |       if ~strcmp(f32RampDown_bkup,tmps)
      |         set_param(gcb,'f32RampDown',tmps);
      |       end
      |     end
      |   end
      | end
      mask Callback wf0:
      | autoCalcEn=get_param(gcb,'autoCalcEn');
      | if strcmp(autoCalcEn,'on')
      |   SampleTime=Simulink.data.evalinGlobal(bdroot,get_param(gcb,'SampleTime'));
      |   if (SampleTime==-1)
      |     SampleTime=str2double(get_param(gcb,'SampleTime_1'));
      |   end
      |   u16NSamplesW_bkup=get_param(gcb,'u16NSamplesW');
      |   u16NSamplesFW_bkup=get_param(gcb,'u16NSamplesFW');
      |   f32PropGainQ_bkup=get_param(gcb,'f32PropGainQ');
      |   f32IntegGainQ_bkup=get_param(gcb,'f32IntegGainQ');
      |   s16PropGainShiftQ_bkup=get_param(gcb,'s16PropGainShiftQ');
      |   s16IntegGainShiftQ_bkup=get_param(gcb,'s16IntegGainShiftQ');
      |   f32LowerLimitQ_bkup=get_param(gcb,'f32LowerLimitQ');
      |   f32UpperLimitQ_bkup=get_param(gcb,'f32UpperLimitQ');
      |   f32PropGainFW_bkup=get_param(gcb,'f32PropGainFW');
      |   f32IntegGainFW_bkup=get_param(gcb,'f32IntegGainFW');
      |   s16PropGainShiftFW_bkup=get_param(gcb,'s16PropGainShiftFW');
      |   s16IntegGainShiftFW_bkup=get_param(gcb,'s16IntegGainShiftFW');
      |   f32LowerLimitFW_bkup=get_param(gcb,'f32LowerLimitFW');
      |   f32UpperLimitFW_bkup=get_param(gcb,'f32UpperLimitFW');
      |   f32RampUp_bkup=get_param(gcb,'f32RampUp');
      |   f32RampDown_bkup=get_param(gcb,'f32RampDown');
      |   wf0=Simulink.data.evalinGlobal(bdroot,get_param(gcb,'wf0'));
      |   wksi=Simulink.data.evalinGlobal(bdroot,get_param(gcb,'wksi'));
      |   J=Simulink.data.evalinGlobal(bdroot,get_param(gcb,'J'));
      |   Kt=Simulink.data.evalinGlobal(bdroot,get_param(gcb,'Kt'));
      |   lambdaW=Simulink.data.evalinGlobal(bdroot,get_param(gcb,'lambdaW'));
      |   lambdaFW=Simulink.data.evalinGlobal(bdroot,get_param(gcb,'lambdaFW'));
      |   Idmax=Simulink.data.evalinGlobal(bdroot,get_param(gcb,'Idmax'));
      |   ramprpm=Simulink.data.evalinGlobal(bdroot,get_param(gcb,'ramprpm'));
      |   mechspeed=Simulink.data.evalinGlobal(bdroot,get_param(gcb,'mechspeed'));
      |   polepairs=Simulink.data.evalinGlobal(bdroot,get_param(gcb,'polepairs'));
      |   uscale=Simulink.data.evalinGlobal(bdroot,get_param(gcb,'uscale'));
      |   iscale=Simulink.data.evalinGlobal(bdroot,get_param(gcb,'iscale'));
      |   if (wf0<=0)
      |     warning('Natural frequency f0 must be positive.');
      |   end
      |   if (wksi<=0)
      |     warning('Current loop attenuation must be positive.');
      |   end
      |   if (wksi>1)
      |     warning('Current loop attenuation must not exceed 1.');
      |   end
      |   if (J<=0)
      |     warning('Moment of inertia J must be positive.');
      |   end
      |   if (Kt<=0)
      |     warning('Torque constant Kt must be positive.');
      |   end
      |   if (lambdaW<0)
      |     warning('MA filter smoothing factor must be in the range 0..1.');
      |   end
      |   if (lambdaW>1)
      |     warning('MA filter smoothing factor must be in the range 0..1.');
      |   end
      |   if (lambdaFW<0)
      |     warning('MA filter smoothing factor must be in the range 0..1.');
      |   end
      |   if (lambdaFW>1)
      |     warning('MA filter smoothing factor must be in the range 0..1.');
      |   end
      |   if (mechspeed<=0)
      |     warning('Max. speed must be positive.');
      |   end
      |   if (polepairs<1)
      |     warning('Number of pole pairs must be a natural number (1, 2, 3, ...).');
      |   end
      |   if (round(polepairs)~=polepairs)
      |     warning('Number of pole pairs must be a natural number (1, 2, 3, ...).');
      |   end
      |   if (uscale<=0)
      |     warning('U_max must be positive.');
      |   end
      |   if (iscale<=0)
      |     warning('I_max must be positive.');
      |   end
      |   w0=6.283185307179586*wf0;
      |   pgain=2.0*wksi*w0*J/Kt;
      |   igain=w0*w0*J/Kt;
      |   wmax=polepairs*mechspeed*0.1047197551196598;
      |   kpf=pgain*wmax/iscale;
      |   s16PropGainShiftQ=ceil(log2(abs(kpf)));
      |   if s16PropGainShiftQ<-31
      |     s16PropGainShiftQ=-31;
      |   end
      |   if s16PropGainShiftQ>31
      |     s16PropGainShiftQ=31;
      |     warning(['Parameter s16PropGainShiftQ of ' gcb ' exceeds the fixed-point range.']);
      |   end
      |   f32PropGainQ=round(kpf*2^(-s16PropGainShiftQ)*2^31);
      |   if f32PropGainQ>2^31-1
      |     f32PropGainQ=2^31-1;
      |     warning(['Parameter f32PropGainQ of ' gcb ' exceeds the fixed-point range.']);
      |   end
      |   if f32PropGainQ<-2^31
      |     f32PropGainQ=-2^31;
      |     warning(['Parameter f32PropGainQ of ' gcb ' exceeds the fixed-point range.']);
      |   end
      |   kif=igain*SampleTime*0.5*wmax/iscale;
      |   s16IntegGainShiftQ=ceil(log2(abs(kif)));
      |   if s16IntegGainShiftQ<-31
      |     s16IntegGainShiftQ=-31;
      |   end
      |   if s16IntegGainShiftQ>31
      |     s16IntegGainShiftQ=31;
      |     warning(['Parameter s16IntegGainShiftQ of ' gcb ' exceeds the fixed-point range.']);
      |   end
      |   f32IntegGainQ=round(kif*2^(-s16IntegGainShiftQ)*2^31);
      |   if f32IntegGainQ>2^31-1
      |     f32IntegGainQ=2^31-1;
      |     warning(['Parameter f32IntegGainQ of ' gcb ' exceeds the fixed-point range.']);
      |   end
      |   if f32IntegGainQ<-2^31
      |     f32IntegGainQ=-2^31;
      |     warning(['Parameter f32IntegGainQ of ' gcb ' exceeds the fixed-point range.']);
      |   end
      |   f32LowerLimitQ=-2147483648;
      |   f32UpperLimitQ=2147483647;
      |   fwkpf=0.9*pgain*wmax/iscale;
      |   s16PropGainShiftFW=ceil(log2(abs(fwkpf)));
      |   if s16PropGainShiftFW<-31
      |     s16PropGainShiftFW=-31;
      |   end
      |   if s16PropGainShiftFW>31
      |     s16PropGainShiftFW=31;
      |     warning(['Parameter s16PropGainShiftFW of ' gcb ' exceeds the fixed-point range.']);
      |   end
      |   f32PropGainFW=round(fwkpf*2^(-s16PropGainShiftFW)*2^31);
      |   if f32PropGainFW>2^31-1
      |     f32PropGainFW=2^31-1;
      |     warning(['Parameter f32PropGainFW of ' gcb ' exceeds the fixed-point range.']);
      |   end
      |   if f32PropGainFW<-2^31
      |     f32PropGainFW=-2^31;
      |     warning(['Parameter f32PropGainFW of ' gcb ' exceeds the fixed-point range.']);
      |   end
      |   s16IntegGainShiftFW=s16IntegGainShiftQ;
      |   f32IntegGainFW=f32IntegGainQ;
      |   if (Idmax<0)
      |     iratio=abs(Idmax)/iscale;
      |     if (abs(iratio) > 1)
      |       iratio = 0;
      |     end
      |     lowlim=0.3183098861837907*acos(iratio)-0.5;
      |   else
      |     lowlim=0.0;
      |   end
      |   f32LowerLimitFW=round(lowlim*2^31);
      |   if f32LowerLimitFW>2^31-1
      |     f32LowerLimitFW=2^31-1;
      |     warning(['Parameter f32LowerLimitFW of ' gcb ' exceeds the fixed-point range.']);
      |   end
      |   if f32LowerLimitFW<-2^31
      |     f32LowerLimitFW=-2^31;
      |     warning(['Parameter f32LowerLimitFW of ' gcb ' exceeds the fixed-point range.']);
      |   end
      |   f32UpperLimitFW=0;
      |   u16NSamplesW=round(log2(1.0/abs(lambdaW)));
      |   if u16NSamplesW>31
      |     u16NSamplesW=31;
      |   end
      |   if u16NSamplesW<0
      |     u16NSamplesW=0;
      |   end
      |   u16NSamplesFW=round(log2(1.0/abs(lambdaFW)));
      |   if u16NSamplesFW>31
      |     u16NSamplesFW=31;
      |   end
      |   if u16NSamplesFW<0
      |     u16NSamplesFW=0;
      |   end
      |   rampsc=polepairs*abs(ramprpm)*0.1047197551196598/wmax;
      |   f32RampUp=round(rampsc*2^31);
      |   if f32RampUp>2^31-1
      |     f32RampUp=2^31-1;
      |     warning(['Parameter f32RampUp of ' gcb ' exceeds the fixed-point range.']);
      |   end
      |   if f32RampUp<-2^31
      |     f32RampUp=-2^31;
      |     warning(['Parameter f32RampUp of ' gcb ' exceeds the fixed-point range.']);
      |   end
      |   f32RampDown=round(rampsc*2^31);
      |   if f32RampDown>2^31-1
      |     f32RampDown=2^31-1;
      |     warning(['Parameter f32RampDown of ' gcb ' exceeds the fixed-point range.']);
      |   end
      |   if f32RampDown<-2^31
      |     f32RampDown=-2^31;
      |     warning(['Parameter f32RampDown of ' gcb ' exceeds the fixed-point range.']);
      |   end
      |   if isnan(u16NSamplesW)
      |     if ~strcmp(u16NSamplesW_bkup,'0')
      |       set_param(gcb,'u16NSamplesW','0');
      |     end
      |   else
      |     tmps=num2str(u16NSamplesW);
      |     if ~strcmp(u16NSamplesW_bkup,tmps)
      |       set_param(gcb,'u16NSamplesW',tmps);
      |     end
      |   end
      |   if isnan(u16NSamplesFW)
      |     if ~strcmp(u16NSamplesFW_bkup,'0')
      |       set_param(gcb,'u16NSamplesFW','0');
      |     end
      |   else
      |     tmps=num2str(u16NSamplesFW);
      |     if ~strcmp(u16NSamplesFW_bkup,tmps)
      |       set_param(gcb,'u16NSamplesFW',tmps);
      |     end
      |   end
      |   if isnan(f32PropGainQ)
      |     if ~strcmp(f32PropGainQ_bkup,'0')
      |       set_param(gcb,'f32PropGainQ','0');
      |     end
      |   else
      |     tmps=num2str(f32PropGainQ);
      |     if ~strcmp(f32PropGainQ_bkup,tmps)
      |       set_param(gcb,'f32PropGainQ',tmps);
      |     end
      |   end
      |   if isnan(f32IntegGainQ)
      |     if ~strcmp(f32IntegGainQ_bkup,'0')
      |       set_param(gcb,'f32IntegGainQ','0');
      |     end
      |   else
      |     tmps=num2str(f32IntegGainQ);
      |     if ~strcmp(f32IntegGainQ_bkup,tmps)
      |       set_param(gcb,'f32IntegGainQ',tmps);
      |     end
      |   end
      |   if isnan(s16PropGainShiftQ)
      |     if ~strcmp(s16PropGainShiftQ_bkup,'0')
      |       set_param(gcb,'s16PropGainShiftQ','0');
      |     end
      |   else
      |     tmps=num2str(s16PropGainShiftQ);
      |     if ~strcmp(s16PropGainShiftQ_bkup,tmps)
      |       set_param(gcb,'s16PropGainShiftQ',tmps);
      |     end
      |   end
      |   if isnan(s16IntegGainShiftQ)
      |     if ~strcmp(s16IntegGainShiftQ_bkup,'0')
      |       set_param(gcb,'s16IntegGainShiftQ','0');
      |     end
      |   else
      |     tmps=num2str(s16IntegGainShiftQ);
      |     if ~strcmp(s16IntegGainShiftQ_bkup,tmps)
      |       set_param(gcb,'s16IntegGainShiftQ',tmps);
      |     end
      |   end
      |   if isnan(f32LowerLimitQ)
      |     if ~strcmp(f32LowerLimitQ_bkup,'0')
      |       set_param(gcb,'f32LowerLimitQ','0');
      |     end
      |   else
      |     tmps=num2str(f32LowerLimitQ);
      |     if ~strcmp(f32LowerLimitQ_bkup,tmps)
      |       set_param(gcb,'f32LowerLimitQ',tmps);
      |     end
      |   end
      |   if isnan(f32UpperLimitQ)
      |     if ~strcmp(f32UpperLimitQ_bkup,'0')
      |       set_param(gcb,'f32UpperLimitQ','0');
      |     end
      |   else
      |     tmps=num2str(f32UpperLimitQ);
      |     if ~strcmp(f32UpperLimitQ_bkup,tmps)
      |       set_param(gcb,'f32UpperLimitQ',tmps);
      |     end
      |   end
      |   if isnan(f32PropGainFW)
      |     if ~strcmp(f32PropGainFW_bkup,'0')
      |       set_param(gcb,'f32PropGainFW','0');
      |     end
      |   else
      |     tmps=num2str(f32PropGainFW);
      |     if ~strcmp(f32PropGainFW_bkup,tmps)
      |       set_param(gcb,'f32PropGainFW',tmps);
      |     end
      |   end
      |   if isnan(f32IntegGainFW)
      |     if ~strcmp(f32IntegGainFW_bkup,'0')
      |       set_param(gcb,'f32IntegGainFW','0');
      |     end
      |   else
      |     tmps=num2str(f32IntegGainFW);
      |     if ~strcmp(f32IntegGainFW_bkup,tmps)
      |       set_param(gcb,'f32IntegGainFW',tmps);
      |     end
      |   end
      |   if isnan(s16PropGainShiftFW)
      |     if ~strcmp(s16PropGainShiftFW_bkup,'0')
      |       set_param(gcb,'s16PropGainShiftFW','0');
      |     end
      |   else
      |     tmps=num2str(s16PropGainShiftFW);
      |     if ~strcmp(s16PropGainShiftFW_bkup,tmps)
      |       set_param(gcb,'s16PropGainShiftFW',tmps);
      |     end
      |   end
      |   if isnan(s16IntegGainShiftFW)
      |     if ~strcmp(s16IntegGainShiftFW_bkup,'0')
      |       set_param(gcb,'s16IntegGainShiftFW','0');
      |     end
      |   else
      |     tmps=num2str(s16IntegGainShiftFW);
      |     if ~strcmp(s16IntegGainShiftFW_bkup,tmps)
      |       set_param(gcb,'s16IntegGainShiftFW',tmps);
      |     end
      |   end
      |   if isnan(f32LowerLimitFW)
      |     if ~strcmp(f32LowerLimitFW_bkup,'0')
      |       set_param(gcb,'f32LowerLimitFW','0');
      |     end
      |   else
      |     tmps=num2str(f32LowerLimitFW);
      |     if ~strcmp(f32LowerLimitFW_bkup,tmps)
      |       set_param(gcb,'f32LowerLimitFW',tmps);
      |     end
      |   end
      |   if isnan(f32UpperLimitFW)
      |     if ~strcmp(f32UpperLimitFW_bkup,'0')
      |       set_param(gcb,'f32UpperLimitFW','0');
      |     end
      |   else
      |     tmps=num2str(f32UpperLimitFW);
      |     if ~strcmp(f32UpperLimitFW_bkup,tmps)
      |       set_param(gcb,'f32UpperLimitFW',tmps);
      |     end
      |   end
      |   if isnan(f32RampUp)
      |     if ~strcmp(f32RampUp_bkup,'0')
      |       set_param(gcb,'f32RampUp','0');
      |     end
      |   else
      |     tmps=num2str(f32RampUp);
      |     if ~strcmp(f32RampUp_bkup,tmps)
      |       set_param(gcb,'f32RampUp',tmps);
      |     end
      |   end
      |   if isnan(f32RampDown)
      |     if ~strcmp(f32RampDown_bkup,'0')
      |       set_param(gcb,'f32RampDown','0');
      |     end
      |   else
      |     tmps=num2str(f32RampDown);
      |     if ~strcmp(f32RampDown_bkup,tmps)
      |       set_param(gcb,'f32RampDown',tmps);
      |     end
      |   end
      | end
      mask Callback wksi:
      | autoCalcEn=get_param(gcb,'autoCalcEn');
      | if strcmp(autoCalcEn,'on')
      |   SampleTime=Simulink.data.evalinGlobal(bdroot,get_param(gcb,'SampleTime'));
      |   if (SampleTime==-1)
      |     SampleTime=str2double(get_param(gcb,'SampleTime_1'));
      |   end
      |   u16NSamplesW_bkup=get_param(gcb,'u16NSamplesW');
      |   u16NSamplesFW_bkup=get_param(gcb,'u16NSamplesFW');
      |   f32PropGainQ_bkup=get_param(gcb,'f32PropGainQ');
      |   f32IntegGainQ_bkup=get_param(gcb,'f32IntegGainQ');
      |   s16PropGainShiftQ_bkup=get_param(gcb,'s16PropGainShiftQ');
      |   s16IntegGainShiftQ_bkup=get_param(gcb,'s16IntegGainShiftQ');
      |   f32LowerLimitQ_bkup=get_param(gcb,'f32LowerLimitQ');
      |   f32UpperLimitQ_bkup=get_param(gcb,'f32UpperLimitQ');
      |   f32PropGainFW_bkup=get_param(gcb,'f32PropGainFW');
      |   f32IntegGainFW_bkup=get_param(gcb,'f32IntegGainFW');
      |   s16PropGainShiftFW_bkup=get_param(gcb,'s16PropGainShiftFW');
      |   s16IntegGainShiftFW_bkup=get_param(gcb,'s16IntegGainShiftFW');
      |   f32LowerLimitFW_bkup=get_param(gcb,'f32LowerLimitFW');
      |   f32UpperLimitFW_bkup=get_param(gcb,'f32UpperLimitFW');
      |   f32RampUp_bkup=get_param(gcb,'f32RampUp');
      |   f32RampDown_bkup=get_param(gcb,'f32RampDown');
      |   wf0=Simulink.data.evalinGlobal(bdroot,get_param(gcb,'wf0'));
      |   wksi=Simulink.data.evalinGlobal(bdroot,get_param(gcb,'wksi'));
      |   J=Simulink.data.evalinGlobal(bdroot,get_param(gcb,'J'));
      |   Kt=Simulink.data.evalinGlobal(bdroot,get_param(gcb,'Kt'));
      |   lambdaW=Simulink.data.evalinGlobal(bdroot,get_param(gcb,'lambdaW'));
      |   lambdaFW=Simulink.data.evalinGlobal(bdroot,get_param(gcb,'lambdaFW'));
      |   Idmax=Simulink.data.evalinGlobal(bdroot,get_param(gcb,'Idmax'));
      |   ramprpm=Simulink.data.evalinGlobal(bdroot,get_param(gcb,'ramprpm'));
      |   mechspeed=Simulink.data.evalinGlobal(bdroot,get_param(gcb,'mechspeed'));
      |   polepairs=Simulink.data.evalinGlobal(bdroot,get_param(gcb,'polepairs'));
      |   uscale=Simulink.data.evalinGlobal(bdroot,get_param(gcb,'uscale'));
      |   iscale=Simulink.data.evalinGlobal(bdroot,get_param(gcb,'iscale'));
      |   if (wf0<=0)
      |     warning('Natural frequency f0 must be positive.');
      |   end
      |   if (wksi<=0)
      |     warning('Current loop attenuation must be positive.');
      |   end
      |   if (wksi>1)
      |     warning('Current loop attenuation must not exceed 1.');
      |   end
      |   if (J<=0)
      |     warning('Moment of inertia J must be positive.');
      |   end
      |   if (Kt<=0)
      |     warning('Torque constant Kt must be positive.');
      |   end
      |   if (lambdaW<0)
      |     warning('MA filter smoothing factor must be in the range 0..1.');
      |   end
      |   if (lambdaW>1)
      |     warning('MA filter smoothing factor must be in the range 0..1.');
      |   end
      |   if (lambdaFW<0)
      |     warning('MA filter smoothing factor must be in the range 0..1.');
      |   end
      |   if (lambdaFW>1)
      |     warning('MA filter smoothing factor must be in the range 0..1.');
      |   end
      |   if (mechspeed<=0)
      |     warning('Max. speed must be positive.');
      |   end
      |   if (polepairs<1)
      |     warning('Number of pole pairs must be a natural number (1, 2, 3, ...).');
      |   end
      |   if (round(polepairs)~=polepairs)
      |     warning('Number of pole pairs must be a natural number (1, 2, 3, ...).');
      |   end
      |   if (uscale<=0)
      |     warning('U_max must be positive.');
      |   end
      |   if (iscale<=0)
      |     warning('I_max must be positive.');
      |   end
      |   w0=6.283185307179586*wf0;
      |   pgain=2.0*wksi*w0*J/Kt;
      |   igain=w0*w0*J/Kt;
      |   wmax=polepairs*mechspeed*0.1047197551196598;
      |   kpf=pgain*wmax/iscale;
      |   s16PropGainShiftQ=ceil(log2(abs(kpf)));
      |   if s16PropGainShiftQ<-31
      |     s16PropGainShiftQ=-31;
      |   end
      |   if s16PropGainShiftQ>31
      |     s16PropGainShiftQ=31;
      |     warning(['Parameter s16PropGainShiftQ of ' gcb ' exceeds the fixed-point range.']);
      |   end
